simulink model "EvilSpagetty"  (R2020b)
settings: Solver=VariableStepAuto  StartTime=0.0  StopTime=3  RelTol=1e-3
(part 2 of 7)

== matlab function EvilSpagetty/Vt1 ==
  data: u1 input; y output; u2 input; u3 input; u4 input; u5 input; u6 input; u7 input; u8 input; u9 input; u10 input
function y = fcn(u1,u2,u3,u4,u5,u6,u7,u8,u9,u10)
theta1=u1;
theta2=u2;
theta3=u3;
theta4=u4;
theta5=u5;
d_theta1=u6;
d_theta2=u7;
d_theta3=u8;
d_theta4=u9;
d_theta5=u10;
Z=[(9004151162956663*d_theta2^2*cos(theta2 + theta3 + theta4 - theta5))/37778931862957161709568 - (6049849466133601*d_theta2^2*sin(theta2))/151115727451828646838272 + (3240011242931075*d_theta2^2*cos(theta2 + theta3 + theta4 - 2*theta5))/73786976294838206464 - (3240011242931075*d_theta2^2*cos(theta2 + theta3 + theta4 + 2*theta5))/73786976294838206464 + (9004151162956663*d_theta3^2*cos(theta2 + theta3 + theta4 - theta5))/37778931862957161709568 + (3240011242931075*d_theta3^2*cos(theta2 + theta3 + theta4 - 2*theta5))/73786976294838206464 - (3240011242931075*d_theta3^2*cos(theta2 + theta3 + theta4 + 2*theta5))/73786976294838206464 + (9004151162956663*d_theta4^2*cos(theta2 + theta3 + theta4 - theta5))/37778931862957161709568 + (3240011242931075*d_theta4^2*cos(theta2 + theta3 + theta4 - 2*theta5))/73786976294838206464 - (3240011242931075*d_theta4^2*cos(theta2 + theta3 + theta4 + 2*theta5))/73786976294838206464 - (9004151162956663*d_theta5^2*cos(theta2 + theta3 + theta4 - theta5))/37778931862957161709568 - (4653258611581729*d_theta2^2*sin(theta2 + theta3 + theta4 - theta5))/73786976294838206464 + (2282168433090971*d_theta2^2*sin(theta2 + theta3 + theta4 - 2*theta5))/37778931862957161709568 + (2282168433090971*d_theta2^2*sin(theta2 + theta3 + theta4 + 2*theta5))/37778931862957161709568 - (4653258611581729*d_theta3^2*sin(theta2 + theta3 + theta4 - theta5))/73786976294838206464 + (2282168433090971*d_theta3^2*sin(theta2 + theta3 + theta4 - 2*theta5))/37778931862957161709568 + (2282168433090971*d_theta3^2*sin(theta2 + theta3 + theta4 + 2*theta5))/37778931862957161709568 - (4653258611581729*d_theta4^2*sin(theta2 + theta3 + theta4 - theta5))/73786976294838206464 + (2282168433090971*d_theta4^2*sin(theta2 + theta3 + theta4 - 2*theta5))/37778931862957161709568 + (2282168433090971*d_theta4^2*sin(theta2 + theta3 + theta4 + 2*theta5))/37778931862957161709568 + (4653258611581729*d_theta5^2*sin(theta2 + theta3 + theta4 - theta5))/73786976294838206464 + (d_theta1*d_theta4)/2787593149816327892691964784081045188247552 + (5959870363491779*d_theta2^2*cos(theta2 - theta5))/4722366482869645213696 - (5959870363491779*d_theta5^2*cos(theta2 - theta5))/4722366482869645213696 - (8313573984755043*d_theta2^2*sin(theta2 - theta5))/18446744073709551616 + (8313573984755043*d_theta5^2*sin(theta2 - theta5))/18446744073709551616 - (2263187056021513*d_theta2^2*cos(theta2 + theta3 + theta4))/18446744073709551616 + (7988070105025833*d_theta2^2*cos(theta2 + theta3 + theta5))/9444732965739290427392 - (2263187056021513*d_theta3^2*cos(theta2 + theta3 + theta4))/18446744073709551616 + (7988070105025833*d_theta3^2*cos(theta2 + theta3 + theta5))/9444732965739290427392 - (2263187056021513*d_theta4^2*cos(theta2 + theta3 + theta4))/18446744073709551616 - (7988070105025833*d_theta5^2*cos(theta2 + theta3 + theta5))/9444732965739290427392 - (8356375065390427*d_theta2^2*sin(theta2 + theta3 + theta4))/9223372036854775808 + (5571380563941847*d_theta2^2*sin(theta2 + theta3 + theta5))/18446744073709551616 - (8356375065390427*d_theta3^2*sin(theta2 + theta3 + theta4))/9223372036854775808 + (5571380563941847*d_theta3^2*sin(theta2 + theta3 + theta5))/18446744073709551616 - (8356375065390427*d_theta4^2*sin(theta2 + theta3 + theta4))/9223372036854775808 - (5571380563941847*d_theta5^2*sin(theta2 + theta3 + theta5))/18446744073709551616 + (7988070105025833*d_theta2^2*cos(theta2 + theta3 - theta5))/9444732965739290427392 + (7988070105025833*d_theta3^2*cos(theta2 + theta3 - theta5))/9444732965739290427392 - (7988070105025833*d_theta5^2*cos(theta2 + theta3 - theta5))/9444732965739290427392 - (5571380563941847*d_theta2^2*sin(theta2 + theta3 - theta5))/18446744073709551616 - (5571380563941847*d_theta3^2*sin(theta2 + theta3 - theta5))/18446744073709551616 + (5571380563941847*d_theta5^2*sin(theta2 + theta3 - theta5))/18446744073709551616 + (9004151162956663*d_theta2^2*cos(theta2 + theta3 + theta4 + theta5))/37778931862957161709568 + (9004151162956663*d_theta3^2*cos(theta2 + theta3 + theta4 + theta5))/37778931862957161709568 + (9004151162956663*d_theta4^2*cos(theta2 + theta3 + theta4 + theta5))/37778931862957161709568 - (9004151162956663*d_theta5^2*cos(theta2 + theta3 + theta4 + theta5))/37778931862957161709568 + (4653258611581729*d_theta2^2*sin(theta2 + theta3 + theta4 + theta5))/73786976294838206464 + (4653258611581729*d_theta3^2*sin(theta2 + theta3 + theta4 + theta5))/73786976294838206464 + (4653258611581729*d_theta4^2*sin(theta2 + theta3 + theta4 + theta5))/73786976294838206464 - (4653258611581729*d_theta5^2*sin(theta2 + theta3 + theta4 + theta5))/73786976294838206464 - (8937783066759625*d_theta2^2*cos(theta2 + theta3))/4611686018427387904 - (8937783066759625*d_theta3^2*cos(theta2 + theta3))/4611686018427387904 + (5959870363491779*d_theta2^2*cos(theta2 + theta5))/4722366482869645213696 - (5959870363491779*d_theta5^2*cos(theta2 + theta5))/4722366482869645213696 - (581180430255771*d_theta2^2*sin(theta2 + theta3))/72057594037927936 - (581180430255771*d_theta3^2*sin(theta2 + theta3))/72057594037927936 + (8313573984755043*d_theta2^2*sin(theta2 + theta5))/18446744073709551616 - (8313573984755043*d_theta5^2*sin(theta2 + theta5))/18446744073709551616 - (5218682484910043*d_theta2^2*cos(theta2))/147573952589676412928 - (7028085605816175*d_theta1*d_theta3*cos(theta3))/590295810358705651712 - (d_theta1*d_theta2*cos(theta5))/5575186299632655785383929568162090376495104 - (d_theta1*d_theta3*cos(theta5))/5575186299632655785383929568162090376495104 - (d_theta1*d_theta4*cos(theta5))/5575186299632655785383929568162090376495104 + (12544169*d_theta1*d_theta2*cos(2*theta3 - 2*theta2 + theta5))/22300745198530623141535718272648361505980416 + (12544169*d_theta1*d_theta2*cos(2*theta2 - 2*theta3 + theta5))/22300745198530623141535718272648361505980416 - (1393797*d_theta1*d_theta2*cos(2*theta2 + 2*theta3 + theta5))/22300745198530623141535718272648361505980416 + (12544169*d_theta1*d_theta2*cos(2*theta4 - 2*theta2 + theta5))/22300745198530623141535718272648361505980416 + (12544169*d_theta1*d_theta2*cos(2*theta2 - 2*theta4 + theta5))/22300745198530623141535718272648361505980416 - (1393797*d_theta1*d_theta2*cos(2*theta2 + 2*theta4 + theta5))/22300745198530623141535718272648361505980416 + (12544169*d_theta1*d_theta3*cos(2*theta3 - 2*theta2 + theta5))/22300745198530623141535718272648361505980416 + (12544169*d_theta1*d_theta3*cos(2*theta2 - 2*theta3 + theta5))/22300745198530623141535718272648361505980416 - (1393797*d_theta1*d_theta3*cos(2*theta2 + 2*theta3 + theta5))/22300745198530623141535718272648361505980416 + (12544169*d_theta1*d_theta3*cos(2*theta4 - 2*theta3 + theta5))/22300745198530623141535718272648361505980416 + (12544169*d_theta1*d_theta3*cos(2*theta3 - 2*theta4 + theta5))/22300745198530623141535718272648361505980416 - (1393797*d_theta1*d_theta3*cos(2*theta3 + 2*theta4 + theta5))/22300745198530623141535718272648361505980416 + (12544169*d_theta1*d_theta4*cos(2*theta4 - 2*theta2 + theta5))/22300745198530623141535718272648361505980416 + (12544169*d_theta1*d_theta4*cos(2*theta2 - 2*theta4 + theta5))/22300745198530623141535718272648361505980416 - (1393797*d_theta1*d_theta4*cos(2*theta2 + 2*theta4 + theta5))/22300745198530623141535718272648361505980416 + (2787593*d_theta1*d_theta5*cos(2*theta2 + 2*theta3 + theta5))/11150372599265311570767859136324180752990208 + (12544169*d_theta1*d_theta4*cos(2*theta4 - 2*theta3 + theta5))/22300745198530623141535718272648361505980416 + (12544169*d_theta1*d_theta4*cos(2*theta3 - 2*theta4 + theta5))/22300745198530623141535718272648361505980416 - (1393797*d_theta1*d_theta4*cos(2*theta3 + 2*theta4 + theta5))/22300745198530623141535718272648361505980416 + (2787593*d_theta1*d_theta5*cos(2*theta2 + 2*theta4 + theta5))/11150372599265311570767859136324180752990208 + (2787593*d_theta1*d_theta5*cos(2*theta3 + 2*theta4 + theta5))/11150372599265311570767859136324180752990208 - (d_theta1*d_theta2*sin(theta4))/696898287454081973172991196020261297061888 - (3257081095467945*d_theta1*d_theta3*sin(theta3))/288230376151711744 - (d_theta1*d_theta3*sin(theta4))/696898287454081973172991196020261297061888 - (7220698343344529*d_theta1*d_theta4*sin(theta4))/2305843009213693952 + (d_theta1*d_theta2*sin(2*theta2 + theta3 - theta4))/1393796574908163946345982392040522594123776 + (d_theta1*d_theta2*sin(2*theta2 - theta3 + theta4))/1393796574908163946345982392040522594123776 - (7220698343344529*d_theta1*d_theta2*sin(2*theta2 + 2*theta3 + theta4))/1152921504606846976 + (7136239*d_theta1*d_theta2*sin(2*theta2 + theta4 - theta5))/5708990770823839524233143877797980545530986496 + (21408715*d_theta1*d_theta2*sin(2*theta2 - theta4 + theta5))/5708990770823839524233143877797980545530986496 - (7220698343344529*d_theta1*d_theta3*sin(2*theta2 + 2*theta3 + theta4))/1152921504606846976 - (7220698343344529*d_theta1*d_theta4*sin(2*theta2 + 2*theta3 + theta4))/2305843009213693952 + (7136239*d_theta1*d_theta3*sin(2*theta3 + theta4 - theta5))/5708990770823839524233143877797980545530986496 + (21408715*d_theta1*d_theta3*sin(2*theta3 - theta4 + theta5))/5708990770823839524233143877797980545530986496 - (3568119*d_theta1*d_theta4*sin(2*theta2 + theta4 - theta5))/2854495385411919762116571938898990272765493248 - (3568119*d_theta1*d_theta4*sin(2*theta3 + theta4 - theta5))/2854495385411919762116571938898990272765493248 + (3568119*d_theta1*d_theta5*sin(2*theta2 + theta4 - theta5))/2854495385411919762116571938898990272765493248 + (3568119*d_theta1*d_theta5*sin(2*theta3 + theta4 - theta5))/2854495385411919762116571938898990272765493248 + (8313573984755043*d_theta1*d_theta2*cos(2*theta2 + theta3 + theta4 + theta5))/9223372036854775808 + (8313573984755043*d_theta1*d_theta3*cos(2*theta2 + theta3 + theta4 + theta5))/18446744073709551616 + (9004151162956663*d_theta2*d_theta3*cos(theta2 + theta3 + theta4 - theta5))/18889465931478580854784 + (8313573984755043*d_theta1*d_theta4*cos(2*theta2 + theta3 + theta4 + theta5))/18446744073709551616 + (3240011242931075*d_theta2*d_theta3*cos(theta2 + theta3 + theta4 - 2*theta5))/36893488147419103232 - (3240011242931075*d_theta2*d_theta3*cos(theta2 + theta3 + theta4 + 2*theta5))/36893488147419103232 + (9004151162956663*d_theta2*d_theta4*cos(theta2 + theta3 + theta4 - theta5))/18889465931478580854784 + (8313573984755043*d_theta1*d_theta5*cos(2*theta2 + theta3 + theta4 + theta5))/18446744073709551616 + (3240011242931075*d_theta2*d_theta4*cos(theta2 + theta3 + theta4 - 2*theta5))/36893488147419103232 - (3240011242931075*d_theta2*d_theta4*cos(theta2 + theta3 + theta4 + 2*theta5))/36893488147419103232 + (9004151162956663*d_theta3*d_theta4*cos(theta2 + theta3 + theta4 - theta5))/18889465931478580854784 - (3240011242931075*d_theta2*d_theta5*cos(theta2 + theta3 + theta4 - 2*theta5))/36893488147419103232 - (3240011242931075*d_theta2*d_theta5*cos(theta2 + theta3 + theta4 + 2*theta5))/36893488147419103232 + (3240011242931075*d_theta3*d_theta4*cos(theta2 + theta3 + theta4 - 2*theta5))/36893488147419103232 - (3240011242931075*d_theta3*d_theta4*cos(theta2 + theta3 + theta4 + 2*theta5))/36893488147419103232 - (3240011242931075*d_theta3*d_theta5*cos(theta2 + theta3 + theta4 - 2*theta5))/36893488147419103232 - (3240011242931075*d_theta3*d_theta5*cos(theta2 + theta3 + theta4 + 2*theta5))/36893488147419103232 - (3240011242931075*d_theta4*d_theta5*cos(theta2 + theta3 + theta4 - 2*theta5))/36893488147419103232 - (3240011242931075*d_theta4*d_theta5*cos(theta2 + theta3 + theta4 + 2*theta5))/36893488147419103232 - (5959870363491779*d_theta1*d_theta2*sin(2*theta2 + theta3 + theta4 + theta5))/2361183241434822606848 - (5959870363491779*d_theta1*d_theta3*sin(2*theta2 + theta3 + theta4 + theta5))/4722366482869645213696 - (4653258611581729*d_theta2*d_theta3*sin(theta2 + theta3 + theta4 - theta5))/36893488147419103232 - (5959870363491779*d_theta1*d_theta4*sin(2*theta2 + theta3 + theta4 + theta5))/4722366482869645213696 + (2282168433090971*d_theta2*d_theta3*sin(theta2 + theta3 + theta4 - 2*theta5))/18889465931478580854784 + (2282168433090971*d_theta2*d_theta3*sin(theta2 + theta3 + theta4 + 2*theta5))/18889465931478580854784 - (4653258611581729*d_theta2*d_theta4*sin(theta2 + theta3 + theta4 - theta5))/36893488147419103232 - (5959870363491779*d_theta1*d_theta5*sin(2*theta2 + theta3 + theta4 + theta5))/4722366482869645213696 + (2282168433090971*d_theta2*d_theta4*sin(theta2 + theta3 + theta4 - 2*theta5))/18889465931478580854784 + (2282168433090971*d_theta2*d_theta4*sin(theta2 + theta3 + theta4 + 2*theta5))/18889465931478580854784 - (4653258611581729*d_theta3*d_theta4*sin(theta2 + theta3 + theta4 - theta5))/36893488147419103232 - (2282168433090971*d_theta2*d_theta5*sin(theta2 + theta3 + theta4 - 2*theta5))/18889465931478580854784 + (2282168433090971*d_theta2*d_theta5*sin(theta2 + theta3 + theta4 + 2*theta5))/18889465931478580854784 + (2282168433090971*d_theta3*d_theta4*sin(theta2 + theta3 + theta4 - 2*theta5))/18889465931478580854784 + (2282168433090971*d_theta3*d_theta4*sin(theta2 + theta3 + theta4 + 2*theta5))/18889465931478580854784 - (2282168433090971*d_theta3*d_theta5*sin(theta2 + theta3 + theta4 - 2*theta5))/18889465931478580854784 + (2282168433090971*d_theta3*d_theta5*sin(theta2 + theta3 + theta4 + 2*theta5))/18889465931478580854784 - (2282168433090971*d_theta4*d_theta5*sin(theta2 + theta3 + theta4 - 2*theta5))/18889465931478580854784 + (2282168433090971*d_theta4*d_theta5*sin(theta2 + theta3 + theta4 + 2*theta5))/18889465931478580854784 - (7028085605816175*d_theta1*d_theta2*cos(2*theta2 + theta3))/295147905179352825856 - (7028085605816175*d_theta1*d_theta3*cos(2*theta2 + theta3))/590295810358705651712 + (2787593*d_theta1*d_theta2*cos(2*theta2 + theta5))/5575186299632655785383929568162090376495104 + (2787593*d_theta1*d_theta3*cos(2*theta3 + theta5))/5575186299632655785383929568162090376495104 + (5571380563941847*d_theta1*d_theta4*cos(theta4 - theta5))/18446744073709551616 + (2787593*d_theta1*d_theta5*cos(2*theta2 + theta5))/11150372599265311570767859136324180752990208 + (2787593*d_theta1*d_theta4*cos(2*theta4 + theta5))/5575186299632655785383929568162090376495104 - (5571380563941847*d_theta1*d_theta5*cos(theta4 - theta5))/18446744073709551616 + (2787593*d_theta1*d_theta5*cos(2*theta3 + theta5))/11150372599265311570767859136324180752990208 + (2787593*d_theta1*d_theta5*cos(2*theta4 + theta5))/11150372599265311570767859136324180752990208 + (d_theta1*d_theta2*cos(2*theta2 - 2*theta3 + 2*theta4 - theta5))/89202980794122492566142873090593446023921664 + (d_theta1*d_theta2*cos(2*theta2 + 2*theta3 - 2*theta4 - theta5))/89202980794122492566142873090593446023921664 + (4653258611581729*d_theta1*d_theta2*cos(2*theta2 + 2*theta3 + 2*theta4 - theta5))/36893488147419103232 - (2282168433090971*d_theta1*d_theta2*cos(2*theta2 + 2*theta3 + 2*theta4 - 2*theta5))/37778931862957161709568 + (2282168433090971*d_theta1*d_theta2*cos(2*theta2 + 2*theta3 + 2*theta4 + 2*theta5))/37778931862957161709568 + (22300745*d_theta1*d_theta3*cos(2*theta2 - 2*theta3 + 2*theta4 - theta5))/44601490397061246283071436545296723011960832 + (d_theta1*d_theta3*cos(2*theta2 + 2*theta3 - 2*theta4 - theta5))/89202980794122492566142873090593446023921664 + (4653258611581729*d_theta1*d_theta3*cos(2*theta2 + 2*theta3 + 2*theta4 - theta5))/36893488147419103232 - (2282168433090971*d_theta1*d_theta3*cos(2*theta2 + 2*theta3 + 2*theta4 - 2*theta5))/37778931862957161709568 + (2282168433090971*d_theta1*d_theta3*cos(2*theta2 + 2*theta3 + 2*theta4 + 2*theta5))/37778931862957161709568 + (d_theta1*d_theta4*cos(2*theta2 - 2*theta3 + 2*theta4 - theta5))/89202980794122492566142873090593446023921664 + (22300745*d_theta1*d_theta4*cos(2*theta2 + 2*theta3 - 2*theta4 - theta5))/44601490397061246283071436545296723011960832 + (4653258611581729*d_theta1*d_theta4*cos(2*theta2 + 2*theta3 + 2*theta4 - theta5))/36893488147419103232 - (2282168433090971*d_theta1*d_theta4*cos(2*theta2 + 2*theta3 + 2*theta4 - 2*theta5))/37778931862957161709568 + (2282168433090971*d_theta1*d_theta4*cos(2*theta2 + 2*theta3 + 2*theta4 + 2*theta5))/37778931862957161709568 - (4653258611581729*d_theta1*d_theta5*cos(2*theta2 + 2*theta3 + 2*theta4 - theta5))/73786976294838206464 + (2282168433090971*d_theta1*d_theta5*cos(2*theta2 + 2*theta3 + 2*theta4 - 2*theta5))/37778931862957161709568 + (2282168433090971*d_theta1*d_theta5*cos(2*theta2 + 2*theta3 + 2*theta4 + 2*theta5))/37778931862957161709568 - (3257081095467945*d_theta1*d_theta2*sin(2*theta2 + theta3))/144115188075855872 + (6968983*d_theta1*d_theta2*sin(2*theta2 + theta4))/1393796574908163946345982392040522594123776 - (3257081095467945*d_theta1*d_theta3*sin(2*theta2 + theta3))/288230376151711744 - (2854495*d_theta1*d_theta2*sin(2*theta2 + theta5))/5708990770823839524233143877797980545530986496 + (6968983*d_theta1*d_theta3*sin(2*theta3 + theta4))/1393796574908163946345982392040522594123776 + (6968983*d_theta1*d_theta4*sin(2*theta2 + theta4))/1393796574908163946345982392040522594123776 - (2854495*d_theta1*d_theta3*sin(2*theta3 + theta5))/5708990770823839524233143877797980545530986496 + (6968983*d_theta1*d_theta4*sin(2*theta3 + theta4))/1393796574908163946345982392040522594123776 + (7988070105025833*d_theta1*d_theta4*sin(theta4 - theta5))/9444732965739290427392 - (2854495*d_theta1*d_theta5*sin(2*theta2 + theta5))/11417981541647679048466287755595961091061972992 - (2854495*d_theta1*d_theta4*sin(2*theta4 + theta5))/5708990770823839524233143877797980545530986496 - (7988070105025833*d_theta1*d_theta5*sin(theta4 - theta5))/9444732965739290427392 - (2854495*d_theta1*d_theta5*sin(2*theta3 + theta5))/11417981541647679048466287755595961091061972992 - (2854495*d_theta1*d_theta5*sin(2*theta4 + theta5))/11417981541647679048466287755595961091061972992 - (2263187056021513*d_theta2*d_theta3*cos(theta2 + theta3 + theta4))/9223372036854775808 + (7988070105025833*d_theta2*d_theta3*cos(theta2 + theta3 + theta5))/4722366482869645213696 - (2263187056021513*d_theta2*d_theta4*cos(theta2 + theta3 + theta4))/9223372036854775808 + (8313573984755043*d_theta1*d_theta3*cos(theta3 + theta4 + theta5))/18446744073709551616 + (1951319518623669*d_theta2*d_theta5*cos(theta2 + theta3 + theta4))/9223372036854775808 - (2263187056021513*d_theta3*d_theta4*cos(theta2 + theta3 + theta4))/9223372036854775808 + (8313573984755043*d_theta1*d_theta4*cos(theta3 + theta4 + theta5))/18446744073709551616 + (1951319518623669*d_theta3*d_theta5*cos(theta2 + theta3 + theta4))/9223372036854775808 + (8313573984755043*d_theta1*d_theta5*cos(theta3 + theta4 + theta5))/18446744073709551616 + (1951319518623669*d_theta4*d_theta5*cos(theta2 + theta3 + theta4))/9223372036854775808 - (d_theta1*d_theta2*sin(2*theta2 + 2*theta3 - theta4 - theta5))/5708990770823839524233143877797980545530986496 + (9004151162956663*d_theta1*d_theta2*sin(2*theta2 + 2*theta3 + 2*theta4 - theta5))/18889465931478580854784 - (d_theta1*d_theta3*sin(2*theta2 + 2*theta3 - theta4 - theta5))/5708990770823839524233143877797980545530986496 - (4460149*d_theta1*d_theta2*sin(2*theta3 - 2*theta2 + 2*theta4 + 2*theta5))/89202980794122492566142873090593446023921664 + (4460149*d_theta1*d_theta2*sin(2*theta2 - 2*theta3 - 2*theta4 + 2*theta5))/89202980794122492566142873090593446023921664 + (3240011242931075*d_theta1*d_theta2*sin(2*theta2 + 2*theta3 + 2*theta4 - 2*theta5))/73786976294838206464 + (3240011242931075*d_theta1*d_theta2*sin(2*theta2 + 2*theta3 + 2*theta4 + 2*theta5))/73786976294838206464 + (9004151162956663*d_theta1*d_theta3*sin(2*theta2 + 2*theta3 + 2*theta4 - theta5))/18889465931478580854784 - (4460149*d_theta1*d_theta3*sin(2*theta2 - 2*theta3 + 2*theta4 - 2*theta5))/89202980794122492566142873090593446023921664 - (4460149*d_theta1*d_theta3*sin(2*theta2 - 2*theta3 + 2*theta4 + 2*theta5))/89202980794122492566142873090593446023921664 + (3240011242931075*d_theta1*d_theta3*sin(2*theta2 + 2*theta3 + 2*theta4 - 2*theta5))/73786976294838206464 + (3240011242931075*d_theta1*d_theta3*sin(2*theta2 + 2*theta3 + 2*theta4 + 2*theta5))/73786976294838206464 + (9004151162956663*d_theta1*d_theta4*sin(2*theta2 + 2*theta3 + 2*theta4 - theta5))/18889465931478580854784 - (4460149*d_theta1*d_theta4*sin(2*theta2 + 2*theta3 - 2*theta4 - 2*theta5))/89202980794122492566142873090593446023921664 - (4460149*d_theta1*d_theta4*sin(2*theta2 + 2*theta3 - 2*theta4 + 2*theta5))/89202980794122492566142873090593446023921664 + (3240011242931075*d_theta1*d_theta4*sin(2*theta2 + 2*theta3 + 2*theta4 - 2*theta5))/73786976294838206464 + (3240011242931075*d_theta1*d_theta4*sin(2*theta2 + 2*theta3 + 2*theta4 + 2*theta5))/73786976294838206464 - (9004151162956663*d_theta1*d_theta5*sin(2*theta2 + 2*theta3 + 2*theta4 - theta5))/37778931862957161709568 - (3240011242931075*d_theta1*d_theta5*sin(2*theta2 + 2*theta3 + 2*theta4 - 2*theta5))/73786976294838206464 + (3240011242931075*d_theta1*d_theta5*sin(2*theta2 + 2*theta3 + 2*theta4 + 2*theta5))/73786976294838206464 - (8356375065390427*d_theta2*d_theta3*sin(theta2 + theta3 + theta4))/4611686018427387904 + (5571380563941847*d_theta2*d_theta3*sin(theta2 + theta3 + theta5))/9223372036854775808 - (8356375065390427*d_theta2*d_theta4*sin(theta2 + theta3 + theta4))/4611686018427387904 - (5959870363491779*d_theta1*d_theta3*sin(theta3 + theta4 + theta5))/4722366482869645213696 - (8356375065390427*d_theta3*d_theta4*sin(theta2 + theta3 + theta4))/4611686018427387904 - (5959870363491779*d_theta1*d_theta4*sin(theta3 + theta4 + theta5))/4722366482869645213696 - (5959870363491779*d_theta1*d_theta5*sin(theta3 + theta4 + theta5))/4722366482869645213696 + (3825825015716409*d_theta1*d_theta2*cos(2*theta2))/73786976294838206464 + (d_theta1*d_theta5*cos(2*theta2))/5708990770823839524233143877797980545530986496 + (d_theta1*d_theta5*cos(2*theta3))/5708990770823839524233143877797980545530986496 + (d_theta1*d_theta5*cos(2*theta4))/5708990770823839524233143877797980545530986496 + (2282168433090971*d_theta1*d_theta5*cos(2*theta5))/18889465931478580854784 - (2695991646372651*d_theta1*d_theta2*cos(2*theta2 + 2*theta3 + 2*theta4))/4611686018427387904 - (1393797*d_theta1*d_theta2*cos(2*theta2 + 2*theta3 - theta5))/22300745198530623141535718272648361505980416 + (5708989*d_theta1*d_theta2*cos(2*theta2 + 2*theta3 - 2*theta5))/91343852333181432387730302044767688728495783936 - (5708989*d_theta1*d_theta2*cos(2*theta2 + 2*theta3 + 2*theta5))/91343852333181432387730302044767688728495783936 - (1393797*d_theta1*d_theta2*cos(2*theta2 + 2*theta4 - theta5))/22300745198530623141535718272648361505980416 - (2695991646372651*d_theta1*d_theta3*cos(2*theta2 + 2*theta3 + 2*theta4))/4611686018427387904 - (1393797*d_theta1*d_theta3*cos(2*theta2 + 2*theta3 - theta5))/22300745198530623141535718272648361505980416 + (5708989*d_theta1*d_theta2*cos(2*theta2 + 2*theta4 - 2*theta5))/91343852333181432387730302044767688728495783936 - (5708989*d_theta1*d_theta2*cos(2*theta2 + 2*theta4 + 2*theta5))/91343852333181432387730302044767688728495783936 + (5708989*d_theta1*d_theta3*cos(2*theta2 + 2*theta3 - 2*theta5))/91343852333181432387730302044767688728495783936 - (5708989*d_theta1*d_theta3*cos(2*theta2 + 2*theta3 + 2*theta5))/91343852333181432387730302044767688728495783936 - (2695991646372651*d_theta1*d_theta4*cos(2*theta2 + 2*theta3 + 2*theta4))/4611686018427387904 - (1393797*d_theta1*d_theta3*cos(2*theta3 + 2*theta4 - theta5))/22300745198530623141535718272648361505980416 - (1393797*d_theta1*d_theta4*cos(2*theta2 + 2*theta4 - theta5))/22300745198530623141535718272648361505980416 - (d_theta1*d_theta5*cos(2*theta3 - 2*theta2 + 2*theta4))/45671926166590716193865151022383844364247891968 - (d_theta1*d_theta5*cos(2*theta2 - 2*theta3 + 2*theta4))/45671926166590716193865151022383844364247891968 - (d_theta1*d_theta5*cos(2*theta2 + 2*theta3 - 2*theta4))/45671926166590716193865151022383844364247891968 - (d_theta1*d_theta5*cos(2*theta2 + 2*theta3 + 2*theta4))/45671926166590716193865151022383844364247891968 - (2787593*d_theta1*d_theta5*cos(2*theta2 + 2*theta3 - theta5))/11150372599265311570767859136324180752990208 + (5708989*d_theta1*d_theta3*cos(2*theta3 + 2*theta4 - 2*theta5))/91343852333181432387730302044767688728495783936 - (5708989*d_theta1*d_theta3*cos(2*theta3 + 2*theta4 + 2*theta5))/91343852333181432387730302044767688728495783936 + (5708989*d_theta1*d_theta4*cos(2*theta2 + 2*theta4 - 2*theta5))/91343852333181432387730302044767688728495783936 - (5708989*d_theta1*d_theta4*cos(2*theta2 + 2*theta4 + 2*theta5))/91343852333181432387730302044767688728495783936 - (1393797*d_theta1*d_theta4*cos(2*theta3 + 2*theta4 - theta5))/22300745198530623141535718272648361505980416 + (d_theta1*d_theta5*cos(2*theta3 - 2*theta2 + 2*theta5))/91343852333181432387730302044767688728495783936 + (d_theta1*d_theta5*cos(2*theta2 - 2*theta3 + 2*theta5))/91343852333181432387730302044767688728495783936 - (2854495*d_theta1*d_theta5*cos(2*theta2 + 2*theta3 - 2*theta5))/45671926166590716193865151022383844364247891968 - (2854495*d_theta1*d_theta5*cos(2*theta2 + 2*theta3 + 2*theta5))/45671926166590716193865151022383844364247891968 - (2787593*d_theta1*d_theta5*cos(2*theta2 + 2*theta4 - theta5))/11150372599265311570767859136324180752990208 + (5708989*d_theta1*d_theta4*cos(2*theta3 + 2*theta4 - 2*theta5))/91343852333181432387730302044767688728495783936 - (5708989*d_theta1*d_theta4*cos(2*theta3 + 2*theta4 + 2*theta5))/91343852333181432387730302044767688728495783936 + (d_theta1*d_theta5*cos(2*theta4 - 2*theta2 + 2*theta5))/91343852333181432387730302044767688728495783936 + (d_theta1*d_theta5*cos(2*theta2 - 2*theta4 + 2*theta5))/91343852333181432387730302044767688728495783936 - (2854495*d_theta1*d_theta5*cos(2*theta2 + 2*theta4 - 2*theta5))/45671926166590716193865151022383844364247891968 - (2854495*d_theta1*d_theta5*cos(2*theta2 + 2*theta4 + 2*theta5))/45671926166590716193865151022383844364247891968 - (2787593*d_theta1*d_theta5*cos(2*theta3 + 2*theta4 - theta5))/11150372599265311570767859136324180752990208 + (d_theta1*d_theta5*cos(2*theta4 - 2*theta3 + 2*theta5))/91343852333181432387730302044767688728495783936 + (d_theta1*d_theta5*cos(2*theta3 - 2*theta4 + 2*theta5))/91343852333181432387730302044767688728495783936 - (2854495*d_theta1*d_theta5*cos(2*theta3 + 2*theta4 - 2*theta5))/45671926166590716193865151022383844364247891968 - (2854495*d_theta1*d_theta5*cos(2*theta3 + 2*theta4 + 2*theta5))/45671926166590716193865151022383844364247891968 - (4725330594848641*d_theta1*d_theta2*sin(2*theta2))/144115188075855872 - (d_theta1*d_theta2*sin(2*theta3))/44601490397061246283071436545296723011960832 - (d_theta1*d_theta3*sin(2*theta2))/44601490397061246283071436545296723011960832 - (d_theta1*d_theta2*sin(2*theta4))/44601490397061246283071436545296723011960832 + (61327049*d_theta1*d_theta3*sin(2*theta3))/44601490397061246283071436545296723011960832 - (d_theta1*d_theta4*sin(2*theta2))/44601490397061246283071436545296723011960832 - (d_theta1*d_theta3*sin(2*theta4))/44601490397061246283071436545296723011960832 - (d_theta1*d_theta4*sin(2*theta3))/44601490397061246283071436545296723011960832 + (61327057*d_theta1*d_theta4*sin(2*theta4))/44601490397061246283071436545296723011960832 + (3240011242931075*d_theta1*d_theta5*sin(2*theta5))/36893488147419103232 - (11150373*d_theta1*d_theta2*sin(2*theta3 - 2*theta2 + 2*theta4))/11150372599265311570767859136324180752990208 - (d_theta1*d_theta2*sin(2*theta2 - 2*theta3 + 2*theta4))/22300745198530623141535718272648361505980416 - (d_theta1*d_theta2*sin(2*theta2 + 2*theta3 - 2*theta4))/22300745198530623141535718272648361505980416 - (1160499590055099*d_theta1*d_theta2*sin(2*theta2 + 2*theta3 + 2*theta4))/2305843009213693952 - (2787593*d_theta1*d_theta2*sin(2*theta3 - 2*theta2 + 2*theta5))/89202980794122492566142873090593446023921664 + (5575185*d_theta1*d_theta2*sin(2*theta2 - 2*theta3 + 2*theta5))/178405961588244985132285746181186892047843328 + (8362779*d_theta1*d_theta2*sin(2*theta2 + 2*theta3 - 2*theta5))/89202980794122492566142873090593446023921664 + (8362779*d_theta1*d_theta2*sin(2*theta2 + 2*theta3 + 2*theta5))/89202980794122492566142873090593446023921664 - (d_theta1*d_theta3*sin(2*theta3 - 2*theta2 + 2*theta4))/22300745198530623141535718272648361505980416 - (11150373*d_theta1*d_theta3*sin(2*theta2 - 2*theta3 + 2*theta4))/11150372599265311570767859136324180752990208 - (d_theta1*d_theta3*sin(2*theta2 + 2*theta3 - 2*theta4))/22300745198530623141535718272648361505980416 - (1160499590055099*d_theta1*d_theta3*sin(2*theta2 + 2*theta3 + 2*theta4))/2305843009213693952 - (2787593*d_theta1*d_theta2*sin(2*theta4 - 2*theta2 + 2*theta5))/89202980794122492566142873090593446023921664 + (5575185*d_theta1*d_theta2*sin(2*theta2 - 2*theta4 + 2*theta5))/178405961588244985132285746181186892047843328 + (8362779*d_theta1*d_theta2*sin(2*theta2 + 2*theta4 - 2*theta5))/89202980794122492566142873090593446023921664 + (8362779*d_theta1*d_theta2*sin(2*theta2 + 2*theta4 + 2*theta5))/89202980794122492566142873090593446023921664 + (5575185*d_theta1*d_theta3*sin(2*theta3 - 2*theta2 + 2*theta5))/178405961588244985132285746181186892047843328 - (2787593*d_theta1*d_theta3*sin(2*theta2 - 2*theta3 + 2*theta5))/89202980794122492566142873090593446023921664 + (8362779*d_theta1*d_theta3*sin(2*theta2 + 2*theta3 - 2*theta5))/89202980794122492566142873090593446023921664 + (8362779*d_theta1*d_theta3*sin(2*theta2 + 2*theta3 + 2*theta5))/89202980794122492566142873090593446023921664 - (d_theta1*d_theta4*sin(2*theta3 - 2*theta2 + 2*theta4))/22300745198530623141535718272648361505980416 - (d_theta1*d_theta4*sin(2*theta2 - 2*theta3 + 2*theta4))/22300745198530623141535718272648361505980416 - (11150373*d_theta1*d_theta4*sin(2*theta2 + 2*theta3 - 2*theta4))/11150372599265311570767859136324180752990208 - (1160499590055099*d_theta1*d_theta4*sin(2*theta2 + 2*theta3 + 2*theta4))/2305843009213693952 - (2787593*d_theta1*d_theta3*sin(2*theta4 - 2*theta3 + 2*theta5))/89202980794122492566142873090593446023921664 + (5575185*d_theta1*d_theta3*sin(2*theta3 - 2*theta4 + 2*theta5))/178405961588244985132285746181186892047843328 + (8362779*d_theta1*d_theta3*sin(2*theta3 + 2*theta4 - 2*theta5))/89202980794122492566142873090593446023921664 + (8362779*d_theta1*d_theta3*sin(2*theta3 + 2*theta4 + 2*theta5))/89202980794122492566142873090593446023921664 + (5575185*d_theta1*d_theta4*sin(2*theta4 - 2*theta2 + 2*theta5))/178405961588244985132285746181186892047843328 - (2787593*d_theta1*d_theta4*sin(2*theta2 - 2*theta4 + 2*theta5))/89202980794122492566142873090593446023921664 + (8362779*d_theta1*d_theta4*sin(2*theta2 + 2*theta4 - 2*theta5))/89202980794122492566142873090593446023921664 + (8362779*d_theta1*d_theta4*sin(2*theta2 + 2*theta4 + 2*theta5))/89202980794122492566142873090593446023921664 - (2787593*d_theta1*d_theta5*sin(2*theta2 + 2*theta3 - 2*theta5))/22300745198530623141535718272648361505980416 + (2787593*d_theta1*d_theta5*sin(2*theta2 + 2*theta3 + 2*theta5))/22300745198530623141535718272648361505980416 + (5575185*d_theta1*d_theta4*sin(2*theta4 - 2*theta3 + 2*theta5))/178405961588244985132285746181186892047843328 - (2787593*d_theta1*d_theta4*sin(2*theta3 - 2*theta4 + 2*theta5))/89202980794122492566142873090593446023921664 + (8362779*d_theta1*d_theta4*sin(2*theta3 + 2*theta4 - 2*theta5))/89202980794122492566142873090593446023921664 + (8362779*d_theta1*d_theta4*sin(2*theta3 + 2*theta4 + 2*theta5))/89202980794122492566142873090593446023921664 - (2787593*d_theta1*d_theta5*sin(2*theta2 + 2*theta4 - 2*theta5))/22300745198530623141535718272648361505980416 + (2787593*d_theta1*d_theta5*sin(2*theta2 + 2*theta4 + 2*theta5))/22300745198530623141535718272648361505980416 - (2787593*d_theta1*d_theta5*sin(2*theta3 + 2*theta4 - 2*theta5))/22300745198530623141535718272648361505980416 + (2787593*d_theta1*d_theta5*sin(2*theta3 + 2*theta4 + 2*theta5))/22300745198530623141535718272648361505980416 + (8313573984755043*d_theta1*d_theta2*cos(2*theta2 + theta3 + theta4 - theta5))/9223372036854775808 + (5571380563941847*d_theta1*d_theta2*cos(2*theta2 + 2*theta3 + theta4 + theta5))/9223372036854775808 + (8313573984755043*d_theta1*d_theta3*cos(2*theta2 + theta3 + theta4 - theta5))/18446744073709551616 + (5571380563941847*d_theta1*d_theta3*cos(2*theta2 + 2*theta3 + theta4 + theta5))/9223372036854775808 + (8313573984755043*d_theta1*d_theta4*cos(2*theta2 + theta3 + theta4 - theta5))/18446744073709551616 + (5571380563941847*d_theta1*d_theta4*cos(2*theta2 + 2*theta3 + theta4 + theta5))/18446744073709551616 - (8313573984755043*d_theta1*d_theta5*cos(2*theta2 + theta3 + theta4 - theta5))/18446744073709551616 + (5571380563941847*d_theta1*d_theta5*cos(2*theta2 + 2*theta3 + theta4 + theta5))/18446744073709551616 + (5959870363491779*d_theta1*d_theta2*sin(2*theta2 + theta3 + theta4 - theta5))/2361183241434822606848 - (d_theta1*d_theta2*sin(2*theta2 - 2*theta3 + theta4 + theta5))/5708990770823839524233143877797980545530986496 - (7988070105025833*d_theta1*d_theta2*sin(2*theta2 + 2*theta3 + theta4 + theta5))/4722366482869645213696 + (5959870363491779*d_theta1*d_theta3*sin(2*theta2 + theta3 + theta4 - theta5))/4722366482869645213696 - (7988070105025833*d_theta1*d_theta3*sin(2*theta2 + 2*theta3 + theta4 + theta5))/4722366482869645213696 + (5959870363491779*d_theta1*d_theta4*sin(2*theta2 + theta3 + theta4 - theta5))/4722366482869645213696 - (7988070105025833*d_theta1*d_theta4*sin(2*theta2 + 2*theta3 + theta4 + theta5))/9444732965739290427392 - (5959870363491779*d_theta1*d_theta5*sin(2*theta2 + theta3 + theta4 - theta5))/4722366482869645213696 - (7988070105025833*d_theta1*d_theta5*sin(2*theta2 + 2*theta3 + theta4 + theta5))/9444732965739290427392 - (1007824040173657*d_theta1*d_theta2*cos(2*theta2 + 2*theta3))/144115188075855872 + (2787593*d_theta1*d_theta2*cos(2*theta2 - theta5))/5575186299632655785383929568162090376495104 - (1007824040173657*d_theta1*d_theta3*cos(2*theta2 + 2*theta3))/144115188075855872 + (d_theta1*d_theta2*cos(2*theta3 - 2*theta5))/45671926166590716193865151022383844364247891968 + (d_theta1*d_theta2*cos(2*theta3 + 2*theta5))/45671926166590716193865151022383844364247891968 + (d_theta1*d_theta3*cos(2*theta2 - 2*theta5))/45671926166590716193865151022383844364247891968 + (d_theta1*d_theta3*cos(2*theta2 + 2*theta5))/45671926166590716193865151022383844364247891968 + (2787593*d_theta1*d_theta3*cos(2*theta3 - theta5))/5575186299632655785383929568162090376495104 + (d_theta1*d_theta2*cos(2*theta4 - 2*theta5))/45671926166590716193865151022383844364247891968 + (d_theta1*d_theta2*cos(2*theta4 + 2*theta5))/45671926166590716193865151022383844364247891968 + (d_theta1*d_theta4*cos(2*theta2 - 2*theta5))/45671926166590716193865151022383844364247891968 + (d_theta1*d_theta4*cos(2*theta2 + 2*theta5))/45671926166590716193865151022383844364247891968 - (2787593*d_theta1*d_theta5*cos(2*theta2 - theta5))/11150372599265311570767859136324180752990208 + (d_theta1*d_theta3*cos(2*theta4 - 2*theta5))/45671926166590716193865151022383844364247891968 + (d_theta1*d_theta3*cos(2*theta4 + 2*theta5))/45671926166590716193865151022383844364247891968 + (d_theta1*d_theta4*cos(2*theta3 - 2*theta5))/45671926166590716193865151022383844364247891968 + (d_theta1*d_theta4*cos(2*theta3 + 2*theta5))/45671926166590716193865151022383844364247891968 + (2787593*d_theta1*d_theta4*cos(2*theta4 - theta5))/5575186299632655785383929568162090376495104 - (8563485*d_theta1*d_theta5*cos(2*theta2 - 2*theta5))/45671926166590716193865151022383844364247891968 - (8563485*d_theta1*d_theta5*cos(2*theta2 + 2*theta5))/45671926166590716193865151022383844364247891968 - (2787593*d_theta1*d_theta5*cos(2*theta3 - theta5))/11150372599265311570767859136324180752990208 - (8563485*d_theta1*d_theta5*cos(2*theta3 - 2*theta5))/45671926166590716193865151022383844364247891968 - (8563485*d_theta1*d_theta5*cos(2*theta3 + 2*theta5))/45671926166590716193865151022383844364247891968 - (2787593*d_theta1*d_theta5*cos(2*theta4 - theta5))/11150372599265311570767859136324180752990208 - (8563485*d_theta1*d_theta5*cos(2*theta4 - 2*theta5))/45671926166590716193865151022383844364247891968 - (8563485*d_theta1*d_theta5*cos(2*theta4 + 2*theta5))/45671926166590716193865151022383844364247891968 + (8356542075167085*d_theta1*d_theta2*sin(2*theta2 + 2*theta3))/1152921504606846976 - (871123*d_theta1*d_theta2*sin(2*theta2 - theta4))/174224571863520493293247799005065324265472 + (61327057*d_theta1*d_theta2*sin(2*theta2 - 2*theta4))/89202980794122492566142873090593446023921664 + (36238715*d_theta1*d_theta2*sin(2*theta2 + 2*theta4))/44601490397061246283071436545296723011960832 + (2854495*d_theta1*d_theta2*sin(2*theta2 - theta5))/5708990770823839524233143877797980545530986496 + (8356542075167085*d_theta1*d_theta3*sin(2*theta2 + 2*theta3))/1152921504606846976 + (5575185*d_theta1*d_theta2*sin(2*theta2 - 2*theta5))/89202980794122492566142873090593446023921664 + (5575185*d_theta1*d_theta2*sin(2*theta2 + 2*theta5))/89202980794122492566142873090593446023921664 - (871123*d_theta1*d_theta3*sin(2*theta3 - theta4))/174224571863520493293247799005065324265472 - (d_theta1*d_theta4*sin(2*theta2 - theta4))/2787593149816327892691964784081045188247552 - (d_theta1*d_theta2*sin(2*theta3 - 2*theta5))/89202980794122492566142873090593446023921664 - (d_theta1*d_theta2*sin(2*theta3 + 2*theta5))/89202980794122492566142873090593446023921664 - (d_theta1*d_theta3*sin(2*theta2 - 2*theta5))/89202980794122492566142873090593446023921664 - (d_theta1*d_theta3*sin(2*theta2 + 2*theta5))/89202980794122492566142873090593446023921664 + (61327057*d_theta1*d_theta3*sin(2*theta3 - 2*theta4))/89202980794122492566142873090593446023921664 + (36238715*d_theta1*d_theta3*sin(2*theta3 + 2*theta4))/44601490397061246283071436545296723011960832 + (2854495*d_theta1*d_theta3*sin(2*theta3 - theta5))/5708990770823839524233143877797980545530986496 - (30663525*d_theta1*d_theta4*sin(2*theta2 - 2*theta4))/44601490397061246283071436545296723011960832 + (36238715*d_theta1*d_theta4*sin(2*theta2 + 2*theta4))/44601490397061246283071436545296723011960832 - (d_theta1*d_theta4*sin(2*theta3 - theta4))/2787593149816327892691964784081045188247552 - (d_theta1*d_theta2*sin(2*theta4 - 2*theta5))/89202980794122492566142873090593446023921664 - (d_theta1*d_theta2*sin(2*theta4 + 2*theta5))/89202980794122492566142873090593446023921664 + (5575185*d_theta1*d_theta3*sin(2*theta3 - 2*theta5))/89202980794122492566142873090593446023921664 + (5575185*d_theta1*d_theta3*sin(2*theta3 + 2*theta5))/89202980794122492566142873090593446023921664 - (d_theta1*d_theta4*sin(2*theta2 - 2*theta5))/89202980794122492566142873090593446023921664 - (d_theta1*d_theta4*sin(2*theta2 + 2*theta5))/89202980794122492566142873090593446023921664 - (30663525*d_theta1*d_theta4*sin(2*theta3 - 2*theta4))/44601490397061246283071436545296723011960832 + (36238715*d_theta1*d_theta4*sin(2*theta3 + 2*theta4))/44601490397061246283071436545296723011960832 - (2854495*d_theta1*d_theta5*sin(2*theta2 - theta5))/11417981541647679048466287755595961091061972992 - (d_theta1*d_theta3*sin(2*theta4 - 2*theta5))/89202980794122492566142873090593446023921664 - (d_theta1*d_theta3*sin(2*theta4 + 2*theta5))/89202980794122492566142873090593446023921664 - (d_theta1*d_theta4*sin(2*theta3 - 2*theta5))/89202980794122492566142873090593446023921664 - (d_theta1*d_theta4*sin(2*theta3 + 2*theta5))/89202980794122492566142873090593446023921664 + (2854495*d_theta1*d_theta4*sin(2*theta4 - theta5))/5708990770823839524233143877797980545530986496 - (2787593*d_theta1*d_theta5*sin(2*theta2 - 2*theta5))/44601490397061246283071436545296723011960832 + (5575185*d_theta1*d_theta5*sin(2*theta2 + 2*theta5))/89202980794122492566142873090593446023921664 - (2854495*d_theta1*d_theta5*sin(2*theta3 - theta5))/11417981541647679048466287755595961091061972992 + (5575185*d_theta1*d_theta4*sin(2*theta4 - 2*theta5))/89202980794122492566142873090593446023921664 + (5575185*d_theta1*d_theta4*sin(2*theta4 + 2*theta5))/89202980794122492566142873090593446023921664 - (2787593*d_theta1*d_theta5*sin(2*theta3 - 2*theta5))/44601490397061246283071436545296723011960832 + (5575185*d_theta1*d_theta5*sin(2*theta3 + 2*theta5))/89202980794122492566142873090593446023921664 - (2854495*d_theta1*d_theta5*sin(2*theta4 - theta5))/11417981541647679048466287755595961091061972992 - (2787593*d_theta1*d_theta5*sin(2*theta4 - 2*theta5))/44601490397061246283071436545296723011960832 + (5575185*d_theta1*d_theta5*sin(2*theta4 + 2*theta5))/89202980794122492566142873090593446023921664 + (7988070105025833*d_theta2*d_theta3*cos(theta2 + theta3 - theta5))/4722366482869645213696 + (8313573984755043*d_theta1*d_theta3*cos(theta3 + theta4 - theta5))/18446744073709551616 + (8313573984755043*d_theta1*d_theta4*cos(theta3 + theta4 - theta5))/18446744073709551616 - (8313573984755043*d_theta1*d_theta5*cos(theta3 + theta4 - theta5))/18446744073709551616 - (6968983*d_theta1*d_theta2*sin(theta3 - 2*theta2 + theta4))/696898287454081973172991196020261297061888 - (5387337053181017*d_theta1*d_theta2*sin(2*theta2 + theta3 + theta4))/576460752303423488 - (5387337053181017*d_theta1*d_theta3*sin(2*theta2 + theta3 + theta4))/1152921504606846976 + (21408715*d_theta1*d_theta2*sin(theta4 - 2*theta2 + theta5))/5708990770823839524233143877797980545530986496 - (446015*d_theta1*d_theta2*sin(2*theta2 + theta4 + theta5))/356811923176489970264571492362373784095686656 - (5387337053181017*d_theta1*d_theta4*sin(2*theta2 + theta3 + theta4))/1152921504606846976 - (5571380563941847*d_theta2*d_theta3*sin(theta2 + theta3 - theta5))/9223372036854775808 + (5959870363491779*d_theta1*d_theta3*sin(theta3 + theta4 - theta5))/4722366482869645213696 + (21408715*d_theta1*d_theta3*sin(theta4 - 2*theta3 + theta5))/5708990770823839524233143877797980545530986496 - (446015*d_theta1*d_theta3*sin(2*theta3 + theta4 + theta5))/356811923176489970264571492362373784095686656 + (5959870363491779*d_theta1*d_theta4*sin(theta3 + theta4 - theta5))/4722366482869645213696 + (3568119*d_theta1*d_theta4*sin(2*theta2 + theta4 + theta5))/2854495385411919762116571938898990272765493248 + (3568119*d_theta1*d_theta4*sin(2*theta3 + theta4 + theta5))/2854495385411919762116571938898990272765493248 - (5959870363491779*d_theta1*d_theta5*sin(theta3 + theta4 - theta5))/4722366482869645213696 + (3568119*d_theta1*d_theta5*sin(2*theta2 + theta4 + theta5))/2854495385411919762116571938898990272765493248 + (3568119*d_theta1*d_theta5*sin(2*theta3 + theta4 + theta5))/2854495385411919762116571938898990272765493248 + (9004151162956663*d_theta2*d_theta3*cos(theta2 + theta3 + theta4 + theta5))/18889465931478580854784 + (9004151162956663*d_theta2*d_theta4*cos(theta2 + theta3 + theta4 + theta5))/18889465931478580854784 + (9004151162956663*d_theta3*d_theta4*cos(theta2 + theta3 + theta4 + theta5))/18889465931478580854784 + (4653258611581729*d_theta2*d_theta3*sin(theta2 + theta3 + theta4 + theta5))/36893488147419103232 + (4653258611581729*d_theta2*d_theta4*sin(theta2 + theta3 + theta4 + theta5))/36893488147419103232 + (4653258611581729*d_theta3*d_theta4*sin(theta2 + theta3 + theta4 + theta5))/36893488147419103232 - (8937783066759625*d_theta2*d_theta3*cos(theta2 + theta3))/2305843009213693952 + (5571380563941847*d_theta1*d_theta4*cos(theta4 + theta5))/18446744073709551616 + (5571380563941847*d_theta1*d_theta5*cos(theta4 + theta5))/18446744073709551616 + (5571380563941847*d_theta1*d_theta2*cos(2*theta2 + 2*theta3 + theta4 - theta5))/9223372036854775808 + (22300745*d_theta1*d_theta2*cos(2*theta3 - 2*theta2 + 2*theta4 + theta5))/44601490397061246283071436545296723011960832 + (22300745*d_theta1*d_theta2*cos(2*theta2 - 2*theta3 - 2*theta4 + theta5))/44601490397061246283071436545296723011960832 + (d_theta1*d_theta2*cos(2*theta2 - 2*theta3 + 2*theta4 + theta5))/89202980794122492566142873090593446023921664 + (d_theta1*d_theta2*cos(2*theta2 + 2*theta3 - 2*theta4 + theta5))/89202980794122492566142873090593446023921664 + (4653258611581729*d_theta1*d_theta2*cos(2*theta2 + 2*theta3 + 2*theta4 + theta5))/36893488147419103232 + (5571380563941847*d_theta1*d_theta3*cos(2*theta2 + 2*theta3 + theta4 - theta5))/9223372036854775808 + (d_theta1*d_theta3*cos(2*theta3 - 2*theta2 + 2*theta4 + theta5))/89202980794122492566142873090593446023921664 + (d_theta1*d_theta3*cos(2*theta2 - 2*theta3 - 2*theta4 + theta5))/89202980794122492566142873090593446023921664 + (22300745*d_theta1*d_theta3*cos(2*theta2 - 2*theta3 + 2*theta4 + theta5))/44601490397061246283071436545296723011960832 + (d_theta1*d_theta3*cos(2*theta2 + 2*theta3 - 2*theta4 + theta5))/89202980794122492566142873090593446023921664 + (4653258611581729*d_theta1*d_theta3*cos(2*theta2 + 2*theta3 + 2*theta4 + theta5))/36893488147419103232 + (5571380563941847*d_theta1*d_theta4*cos(2*theta2 + 2*theta3 + theta4 - theta5))/18446744073709551616 + (d_theta1*d_theta4*cos(2*theta3 - 2*theta2 + 2*theta4 + theta5))/89202980794122492566142873090593446023921664 + (d_theta1*d_theta4*cos(2*theta2 - 2*theta3 - 2*theta4 + theta5))/89202980794122492566142873090593446023921664 + (d_theta1*d_theta4*cos(2*theta2 - 2*theta3 + 2*theta4 + theta5))/89202980794122492566142873090593446023921664 + (22300745*d_theta1*d_theta4*cos(2*theta2 + 2*theta3 - 2*theta4 + theta5))/44601490397061246283071436545296723011960832 + (4653258611581729*d_theta1*d_theta4*cos(2*theta2 + 2*theta3 + 2*theta4 + theta5))/36893488147419103232 - (5571380563941847*d_theta1*d_theta5*cos(2*theta2 + 2*theta3 + theta4 - theta5))/18446744073709551616 + (4653258611581729*d_theta1*d_theta5*cos(2*theta2 + 2*theta3 + 2*theta4 + theta5))/73786976294838206464 - (581180430255771*d_theta2*d_theta3*sin(theta2 + theta3))/36028797018963968 - (5387337053181017*d_theta1*d_theta3*sin(theta3 + theta4))/1152921504606846976 - (5387337053181017*d_theta1*d_theta4*sin(theta3 + theta4))/1152921504606846976 - (7988070105025833*d_theta1*d_theta4*sin(theta4 + theta5))/9444732965739290427392 - (7988070105025833*d_theta1*d_theta5*sin(theta4 + theta5))/9444732965739290427392 - (d_theta1*d_theta2*sin(2*theta2 - 2*theta3 + theta4 - theta5))/5708990770823839524233143877797980545530986496 + (7988070105025833*d_theta1*d_theta2*sin(2*theta2 + 2*theta3 + theta4 - theta5))/4722366482869645213696 - (d_theta1*d_theta2*sin(2*theta2 + 2*theta3 - theta4 + theta5))/5708990770823839524233143877797980545530986496 - (9004151162956663*d_theta1*d_theta2*sin(2*theta2 + 2*theta3 + 2*theta4 + theta5))/18889465931478580854784 + (7988070105025833*d_theta1*d_theta3*sin(2*theta2 + 2*theta3 + theta4 - theta5))/4722366482869645213696 - (d_theta1*d_theta3*sin(2*theta2 + 2*theta3 - theta4 + theta5))/5708990770823839524233143877797980545530986496 - (9004151162956663*d_theta1*d_theta3*sin(2*theta2 + 2*theta3 + 2*theta4 + theta5))/18889465931478580854784 + (7988070105025833*d_theta1*d_theta4*sin(2*theta2 + 2*theta3 + theta4 - theta5))/9444732965739290427392 - (9004151162956663*d_theta1*d_theta4*sin(2*theta2 + 2*theta3 + 2*theta4 + theta5))/18889465931478580854784 - (7988070105025833*d_theta1*d_theta5*sin(2*theta2 + 2*theta3 + theta4 - theta5))/9444732965739290427392 - (9004151162956663*d_theta1*d_theta5*sin(2*theta2 + 2*theta3 + 2*theta4 + theta5))/37778931862957161709568;
   (d_theta1^2*sin(theta4))/1393796574908163946345982392040522594123776 - (d_theta1^2*sin(theta5))/5708990770823839524233143877797980545530986496 - (3257081095467945*d_theta3^2*sin(theta3))/288230376151711744 - (7220698343344529*d_theta4^2*sin(theta4))/2305843009213693952 - (9004151162956663*d_theta5^2*sin(theta5))/18889465931478580854784 - (3825825015716409*d_theta1^2*cos(2*theta2))/147573952589676412928 + (4725330594848641*d_theta1^2*sin(2*theta2))/288230376151711744 - (d_theta1^2*cos(theta5))/11150372599265311570767859136324180752990208 - (7028085605816175*d_theta3^2*cos(theta3))/590295810358705651712 + (4653258611581729*d_theta5^2*cos(theta5))/36893488147419103232 - (7028085605816175*d_theta2*d_theta3*cos(theta3))/295147905179352825856 - (3257081095467945*d_theta2*d_theta3*sin(theta3))/144115188075855872 - (7220698343344529*d_theta2*d_theta4*sin(theta4))/1152921504606846976 - (7220698343344529*d_theta3*d_theta4*sin(theta4))/1152921504606846976 + (7028085605816175*d_theta1^2*cos(2*theta2)*cos(theta3))/590295810358705651712 + (3257081095467945*d_theta1^2*cos(2*theta2)*sin(theta3))/288230376151711744 + (3257081095467945*d_theta1^2*sin(2*theta2)*cos(theta3))/288230376151711744 - (13937965*d_theta1^2*cos(2*theta2)*sin(theta4))/2787593149816327892691964784081045188247552 - (13937965*d_theta1^2*sin(2*theta2)*cos(theta4))/2787593149816327892691964784081045188247552 - (2854495*d_theta1^2*cos(2*theta2)*sin(theta5))/5708990770823839524233143877797980545530986496 - (7028085605816175*d_theta1^2*sin(2*theta2)*sin(theta3))/590295810358705651712 - (2282168433090971*d_theta2*d_theta5*cos(2*theta5))/9444732965739290427392 - (2282168433090971*d_theta3*d_theta5*cos(2*theta5))/9444732965739290427392 - (2282168433090971*d_theta4*d_theta5*cos(2*theta5))/9444732965739290427392 - (3240011242931075*d_theta2*d_theta5*sin(2*theta5))/18446744073709551616 - (3240011242931075*d_theta3*d_theta5*sin(2*theta5))/18446744073709551616 - (3240011242931075*d_theta4*d_theta5*sin(2*theta5))/18446744073709551616 + (1007824040173657*d_theta1^2*cos(2*theta2)*cos(2*theta3))/288230376151711744 - (d_theta1^2*cos(2*theta2)*cos(2*theta5))/91343852333181432387730302044767688728495783936 - (8356542075167085*d_theta1^2*cos(2*theta2)*sin(2*theta3))/2305843009213693952 - (8356542075167085*d_theta1^2*cos(2*theta3)*sin(2*theta2))/2305843009213693952 + (2787593*d_theta1^2*cos(2*theta2)*sin(2*theta4))/5575186299632655785383929568162090376495104 - (1393797*d_theta1^2*cos(2*theta4)*sin(2*theta2))/22300745198530623141535718272648361505980416 - (1393797*d_theta1^2*cos(2*theta5)*sin(2*theta2))/22300745198530623141535718272648361505980416 - (1007824040173657*d_theta1^2*sin(2*theta2)*sin(2*theta3))/288230376151711744 - (17126969*d_theta1^2*sin(2*theta2)*sin(2*theta5))/91343852333181432387730302044767688728495783936 + (5571380563941847*d_theta4^2*cos(theta4)*cos(theta5))/9223372036854775808 + (5571380563941847*d_theta5^2*cos(theta4)*cos(theta5))/9223372036854775808 - (5387337053181017*d_theta3^2*cos(theta3)*sin(theta4))/1152921504606846976 - (5387337053181017*d_theta3^2*cos(theta4)*sin(theta3))/1152921504606846976 - (5387337053181017*d_theta4^2*cos(theta3)*sin(theta4))/1152921504606846976 - (5387337053181017*d_theta4^2*cos(theta4)*sin(theta3))/1152921504606846976 - (7988070105025833*d_theta4^2*cos(theta4)*sin(theta5))/4722366482869645213696 - (7988070105025833*d_theta5^2*cos(theta4)*sin(theta5))/4722366482869645213696 + (5387337053181017*d_theta1^2*cos(2*theta2)*cos(theta3)*sin(theta4))/1152921504606846976 + (5387337053181017*d_theta1^2*cos(2*theta2)*cos(theta4)*sin(theta3))/1152921504606846976 + (5387337053181017*d_theta1^2*sin(2*theta2)*cos(theta3)*cos(theta4))/1152921504606846976 - (5387337053181017*d_theta1^2*sin(2*theta2)*sin(theta3)*sin(theta4))/1152921504606846976 + (3568119*d_theta1^2*sin(2*theta2)*sin(theta4)*sin(theta5))/1427247692705959881058285969449495136382746624 + (7220698343344529*d_theta1^2*cos(2*theta2)*cos(2*theta3)*sin(theta4))/2305843009213693952 + (7220698343344529*d_theta1^2*cos(2*theta2)*sin(2*theta3)*cos(theta4))/2305843009213693952 + (7220698343344529*d_theta1^2*cos(2*theta3)*sin(2*theta2)*cos(theta4))/2305843009213693952 - (2854495*d_theta1^2*cos(2*theta2)*cos(2*theta3)*sin(theta5))/5708990770823839524233143877797980545530986496 - (2854495*d_theta1^2*cos(2*theta2)*cos(2*theta4)*sin(theta5))/5708990770823839524233143877797980545530986496 + (2787593*d_theta1^2*sin(2*theta2)*sin(2*theta3)*cos(theta5))/5575186299632655785383929568162090376495104 + (2787593*d_theta1^2*sin(2*theta2)*sin(2*theta4)*cos(theta5))/5575186299632655785383929568162090376495104 - (7220698343344529*d_theta1^2*sin(2*theta2)*sin(2*theta3)*sin(theta4))/2305843009213693952 + (8313573984755043*d_theta3^2*cos(theta3)*cos(theta4)*cos(theta5))/9223372036854775808 + (8313573984755043*d_theta4^2*cos(theta3)*cos(theta4)*cos(theta5))/9223372036854775808 + (8313573984755043*d_theta5^2*cos(theta3)*cos(theta4)*cos(theta5))/9223372036854775808 - (5959870363491779*d_theta3^2*cos(theta3)*cos(theta4)*sin(theta5))/2361183241434822606848 - (5959870363491779*d_theta4^2*cos(theta3)*cos(theta4)*sin(theta5))/2361183241434822606848 - (5959870363491779*d_theta5^2*cos(theta3)*cos(theta4)*sin(theta5))/2361183241434822606848 + (2695991646372651*d_theta1^2*cos(2*theta2)*cos(2*theta3)*cos(2*theta4))/9223372036854775808 - (8313573984755043*d_theta3^2*cos(theta5)*sin(theta3)*sin(theta4))/9223372036854775808 - (8313573984755043*d_theta4^2*cos(theta5)*sin(theta3)*sin(theta4))/9223372036854775808 - (8313573984755043*d_theta5^2*cos(theta5)*sin(theta3)*sin(theta4))/9223372036854775808 + (5571380563941847*d_theta2*d_theta4*cos(theta4)*cos(theta5))/4611686018427387904 + (5571380563941847*d_theta3*d_theta4*cos(theta4)*cos(theta5))/4611686018427387904 + (1160499590055099*d_theta1^2*cos(2*theta2)*cos(2*theta3)*sin(2*theta4))/4611686018427387904 + (1160499590055099*d_theta1^2*cos(2*theta2)*cos(2*theta4)*sin(2*theta3))/4611686018427387904 + (1160499590055099*d_theta1^2*cos(2*theta3)*cos(2*theta4)*sin(2*theta2))/4611686018427387904 - (d_theta1^2*cos(2*theta2)*cos(2*theta3)*sin(2*theta5))/356811923176489970264571492362373784095686656 - (d_theta1^2*cos(2*theta2)*cos(2*theta5)*sin(2*theta3))/356811923176489970264571492362373784095686656 - (22300751*d_theta1^2*cos(2*theta3)*cos(2*theta5)*sin(2*theta2))/356811923176489970264571492362373784095686656 - (d_theta1^2*cos(2*theta2)*cos(2*theta4)*sin(2*theta5))/356811923176489970264571492362373784095686656 - (d_theta1^2*cos(2*theta2)*cos(2*theta5)*sin(2*theta4))/356811923176489970264571492362373784095686656 - (22300751*d_theta1^2*cos(2*theta4)*cos(2*theta5)*sin(2*theta2))/356811923176489970264571492362373784095686656 + (5959870363491779*d_theta3^2*sin(theta3)*sin(theta4)*sin(theta5))/2361183241434822606848 + (5959870363491779*d_theta4^2*sin(theta3)*sin(theta4)*sin(theta5))/2361183241434822606848 + (5959870363491779*d_theta5^2*sin(theta3)*sin(theta4)*sin(theta5))/2361183241434822606848 - (5387337053181017*d_theta2*d_theta3*cos(theta3)*sin(theta4))/576460752303423488 - (5387337053181017*d_theta2*d_theta3*cos(theta4)*sin(theta3))/576460752303423488 + (8313573984755043*d_theta1*d_theta5*cos(theta5)*sin(theta2))/4611686018427387904 - (5387337053181017*d_theta2*d_theta4*cos(theta3)*sin(theta4))/576460752303423488 - (5387337053181017*d_theta2*d_theta4*cos(theta4)*sin(theta3))/576460752303423488 - (5387337053181017*d_theta3*d_theta4*cos(theta3)*sin(theta4))/576460752303423488 - (5387337053181017*d_theta3*d_theta4*cos(theta4)*sin(theta3))/576460752303423488 - (7988070105025833*d_theta2*d_theta4*cos(theta4)*sin(theta5))/2361183241434822606848 - (7988070105025833*d_theta2*d_theta5*cos(theta5)*sin(theta4))/2361183241434822606848 - (7988070105025833*d_theta3*d_theta4*cos(theta4)*sin(theta5))/2361183241434822606848 - (7988070105025833*d_theta3*d_theta5*cos(theta5)*sin(theta4))/2361183241434822606848 - (7988070105025833*d_theta4*d_theta5*cos(theta5)*sin(theta4))/2361183241434822606848 - (2695991646372651*d_theta1^2*cos(2*theta2)*sin(2*theta3)*sin(2*theta4))/9223372036854775808 - (2695991646372651*d_theta1^2*cos(2*theta3)*sin(2*theta2)*sin(2*theta4))/9223372036854775808 - (2695991646372651*d_theta1^2*cos(2*theta4)*sin(2*theta2)*sin(2*theta3))/9223372036854775808 + (11417979*d_theta1^2*cos(2*theta2)*sin(2*theta3)*sin(2*theta5))/91343852333181432387730302044767688728495783936 - (2854495*d_theta1^2*cos(2*theta3)*sin(2*theta2)*sin(2*theta5))/45671926166590716193865151022383844364247891968 - (d_theta1^2*cos(2*theta5)*sin(2*theta2)*sin(2*theta3))/91343852333181432387730302044767688728495783936 + (11417979*d_theta1^2*cos(2*theta2)*sin(2*theta4)*sin(2*theta5))/91343852333181432387730302044767688728495783936 - (2854495*d_theta1^2*cos(2*theta4)*sin(2*theta2)*sin(2*theta5))/45671926166590716193865151022383844364247891968 - (d_theta1^2*cos(2*theta5)*sin(2*theta2)*sin(2*theta4))/91343852333181432387730302044767688728495783936 - (5959870363491779*d_theta1*d_theta5*sin(theta2)*sin(theta5))/1180591620717411303424 - (5571380563941847*d_theta2*d_theta5*sin(theta4)*sin(theta5))/4611686018427387904 - (5571380563941847*d_theta3*d_theta5*sin(theta4)*sin(theta5))/4611686018427387904 - (5571380563941847*d_theta4*d_theta5*sin(theta4)*sin(theta5))/4611686018427387904 - (1160499590055099*d_theta1^2*sin(2*theta2)*sin(2*theta3)*sin(2*theta4))/4611686018427387904 - (d_theta1^2*sin(2*theta2)*sin(2*theta3)*sin(2*theta5))/356811923176489970264571492362373784095686656 - (d_theta1^2*sin(2*theta2)*sin(2*theta4)*sin(2*theta5))/356811923176489970264571492362373784095686656 + (10050494243446848990263944093682850882789*d_theta1^2*cos(2*theta2)*cos(theta5)*sin(theta3)*sin(theta4))/11150372599265311570767859136324180752990208 + (10050494243446848990263944093682862033161*d_theta1^2*sin(2*theta2)*cos(theta3)*cos(theta5)*sin(theta4))/11150372599265311570767859136324180752990208 + (10050494243446848990263944093682862033161*d_theta1^2*sin(2*theta2)*cos(theta4)*cos(theta5)*sin(theta3))/11150372599265311570767859136324180752990208 - (3240011242931075*d_theta1^2*cos(2*theta2)*cos(2*theta3)*cos(2*theta5)*sin(2*theta4))/73786976294838206464 - (3240011242931075*d_theta1^2*cos(2*theta2)*cos(2*theta4)*cos(2*theta5)*sin(2*theta3))/73786976294838206464 - (3240011242931075*d_theta1^2*cos(2*theta3)*cos(2*theta4)*cos(2*theta5)*sin(2*theta2))/73786976294838206464 - (5959870363491779*d_theta1^2*cos(2*theta2)*sin(theta3)*sin(theta4)*sin(theta5))/2361183241434822606848 - (5959870363491779*d_theta1^2*sin(2*theta2)*cos(theta3)*sin(theta4)*sin(theta5))/2361183241434822606848 - (5959870363491779*d_theta1^2*sin(2*theta2)*cos(theta4)*sin(theta3)*sin(theta5))/2361183241434822606848 + (2282168433090971*d_theta1^2*cos(2*theta2)*cos(2*theta3)*sin(2*theta4)*sin(2*theta5))/37778931862957161709568 + (2282168433090971*d_theta1^2*cos(2*theta2)*cos(2*theta4)*sin(2*theta3)*sin(2*theta5))/37778931862957161709568 + (2282168433090971*d_theta1^2*cos(2*theta3)*cos(2*theta4)*sin(2*theta2)*sin(2*theta5))/37778931862957161709568 + (3240011242931075*d_theta1^2*cos(2*theta5)*sin(2*theta2)*sin(2*theta3)*sin(2*theta4))/73786976294838206464 - (2282168433090971*d_theta1^2*sin(2*theta2)*sin(2*theta3)*sin(2*theta4)*sin(2*theta5))/37778931862957161709568 - (5571380563941847*d_theta1^2*cos(2*theta2)*cos(2*theta3)*cos(theta4)*cos(theta5))/9223372036854775808 + (7988070105025833*d_theta1^2*cos(2*theta2)*cos(2*theta3)*cos(theta4)*sin(theta5))/4722366482869645213696 + (5571380563941847*d_theta1^2*cos(2*theta2)*sin(2*theta3)*cos(theta5)*sin(theta4))/9223372036854775808 + (5571380563941847*d_theta1^2*cos(2*theta3)*sin(2*theta2)*cos(theta5)*sin(theta4))/9223372036854775808 + (5571380563941847*d_theta1^2*sin(2*theta2)*sin(2*theta3)*cos(theta4)*cos(theta5))/9223372036854775808 - (7988070105025833*d_theta1^2*cos(2*theta2)*sin(2*theta3)*sin(theta4)*sin(theta5))/4722366482869645213696 - (7988070105025833*d_theta1^2*cos(2*theta3)*sin(2*theta2)*sin(theta4)*sin(theta5))/4722366482869645213696 - (7988070105025833*d_theta1^2*sin(2*theta2)*sin(2*theta3)*cos(theta4)*sin(theta5))/4722366482869645213696 - (4653258611581729*d_theta1^2*cos(2*theta2)*cos(2*theta3)*cos(2*theta4)*cos(theta5))/36893488147419103232 - (1951319518623669*d_theta1*d_theta5*cos(theta2)*cos(theta3)*cos(theta4))/9223372036854775808 + (8313573984755043*d_theta2*d_theta3*cos(theta3)*cos(theta4)*cos(theta5))/4611686018427387904 + (8313573984755043*d_theta2*d_theta4*cos(theta3)*cos(theta4)*cos(theta5))/4611686018427387904 + (8313573984755043*d_theta3*d_theta4*cos(theta3)*cos(theta4)*cos(theta5))/4611686018427387904 + (9004151162956663*d_theta1^2*cos(2*theta2)*cos(2*theta3)*cos(2*theta4)*sin(theta5))/18889465931478580854784 + (5571380563941847*d_theta1*d_theta5*cos(theta2)*cos(theta5)*sin(theta3))/4611686018427387904 + (5571380563941847*d_theta1*d_theta5*cos(theta3)*cos(theta5)*sin(theta2))/4611686018427387904 - (5959870363491779*d_theta2*d_theta3*cos(theta3)*cos(theta4)*sin(theta5))/1180591620717411303424 - (5959870363491779*d_theta2*d_theta4*cos(theta3)*cos(theta4)*sin(theta5))/1180591620717411303424 - (5959870363491779*d_theta2*d_theta5*cos(theta3)*cos(theta5)*sin(theta4))/1180591620717411303424 - (5959870363491779*d_theta2*d_theta5*cos(theta4)*cos(theta5)*sin(theta3))/1180591620717411303424 - (5959870363491779*d_theta3*d_theta4*cos(theta3)*cos(theta4)*sin(theta5))/1180591620717411303424 - (5959870363491779*d_theta3*d_theta5*cos(theta3)*cos(theta5)*sin(theta4))/1180591620717411303424 - (5959870363491779*d_theta3*d_theta5*cos(theta4)*cos(theta5)*sin(theta3))/1180591620717411303424 - (5959870363491779*d_theta4*d_theta5*cos(theta3)*cos(theta5)*sin(theta4))/1180591620717411303424 - (5959870363491779*d_theta4*d_theta5*cos(theta4)*cos(theta5)*sin(theta3))/1180591620717411303424 + (4653258611581729*d_theta1^2*cos(2*theta2)*sin(2*theta3)*sin(2*theta4)*cos(theta5))/36893488147419103232 + (4653258611581729*d_theta1^2*cos(2*theta3)*sin(2*theta2)*sin(2*theta4)*cos(theta5))/36893488147419103232 + (4653258611581729*d_theta1^2*cos(2*theta4)*sin(2*theta2)*sin(2*theta3)*cos(theta5))/36893488147419103232 + (1951319518623669*d_theta1*d_theta5*cos(theta2)*sin(theta3)*sin(theta4))/9223372036854775808 + (1951319518623669*d_theta1*d_theta5*cos(theta3)*sin(theta2)*sin(theta4))/9223372036854775808 + (1951319518623669*d_theta1*d_theta5*cos(theta4)*sin(theta2)*sin(theta3))/9223372036854775808 - (7988070105025833*d_theta1*d_theta5*cos(theta2)*sin(theta3)*sin(theta5))/2361183241434822606848 - (7988070105025833*d_theta1*d_theta5*cos(theta3)*sin(theta2)*sin(theta5))/2361183241434822606848 - (8313573984755043*d_theta2*d_theta3*cos(theta5)*sin(theta3)*sin(theta4))/4611686018427387904 - (8313573984755043*d_theta2*d_theta4*cos(theta5)*sin(theta3)*sin(theta4))/4611686018427387904 - (8313573984755043*d_theta2*d_theta5*cos(theta3)*sin(theta4)*sin(theta5))/4611686018427387904 - (8313573984755043*d_theta2*d_theta5*cos(theta4)*sin(theta3)*sin(theta5))/4611686018427387904 - (8313573984755043*d_theta3*d_theta4*cos(theta5)*sin(theta3)*sin(theta4))/4611686018427387904 - (8313573984755043*d_theta3*d_theta5*cos(theta3)*sin(theta4)*sin(theta5))/4611686018427387904 - (8313573984755043*d_theta3*d_theta5*cos(theta4)*sin(theta3)*sin(theta5))/4611686018427387904 - (8313573984755043*d_theta4*d_theta5*cos(theta3)*sin(theta4)*sin(theta5))/4611686018427387904 - (8313573984755043*d_theta4*d_theta5*cos(theta4)*sin(theta3)*sin(theta5))/4611686018427387904 - (9004151162956663*d_theta1^2*cos(2*theta2)*sin(2*theta3)*sin(2*theta4)*sin(theta5))/18889465931478580854784 - (9004151162956663*d_theta1^2*cos(2*theta3)*sin(2*theta2)*sin(2*theta4)*sin(theta5))/18889465931478580854784 - (9004151162956663*d_theta1^2*cos(2*theta4)*sin(2*theta2)*sin(2*theta3)*sin(theta5))/18889465931478580854784 + (5959870363491779*d_theta2*d_theta3*sin(theta3)*sin(theta4)*sin(theta5))/1180591620717411303424 + (5959870363491779*d_theta2*d_theta4*sin(theta3)*sin(theta4)*sin(theta5))/1180591620717411303424 + (5959870363491779*d_theta3*d_theta4*sin(theta3)*sin(theta4)*sin(theta5))/1180591620717411303424 - (10050494243446848990263944093682862033161*d_theta1^2*cos(2*theta2)*cos(theta3)*cos(theta4)*cos(theta5))/11150372599265311570767859136324180752990208 + (5959870363491779*d_theta1^2*cos(2*theta2)*cos(theta3)*cos(theta4)*sin(theta5))/2361183241434822606848 + (3240011242931075*d_theta1*d_theta5*cos(2*theta5)*cos(theta2)*sin(theta3)*sin(theta4))/18446744073709551616 + (3240011242931075*d_theta1*d_theta5*cos(2*theta5)*cos(theta3)*sin(theta2)*sin(theta4))/18446744073709551616 + (3240011242931075*d_theta1*d_theta5*cos(2*theta5)*cos(theta4)*sin(theta2)*sin(theta3))/18446744073709551616 - (2282168433090971*d_theta1*d_theta5*sin(2*theta5)*cos(theta2)*sin(theta3)*sin(theta4))/9444732965739290427392 - (2282168433090971*d_theta1*d_theta5*sin(2*theta5)*cos(theta3)*sin(theta2)*sin(theta4))/9444732965739290427392 - (2282168433090971*d_theta1*d_theta5*sin(2*theta5)*cos(theta4)*sin(theta2)*sin(theta3))/9444732965739290427392 + (4653258611581729*d_theta1*d_theta5*cos(theta2)*cos(theta3)*cos(theta5)*sin(theta4))/18446744073709551616 + (4653258611581729*d_theta1*d_theta5*cos(theta2)*cos(theta4)*cos(theta5)*sin(theta3))/18446744073709551616 + (4653258611581729*d_theta1*d_theta5*cos(theta3)*cos(theta4)*cos(theta5)*sin(theta2))/18446744073709551616 - (9004151162956663*d_theta1*d_theta5*cos(theta2)*cos(theta3)*sin(theta4)*sin(theta5))/9444732965739290427392 - (9004151162956663*d_theta1*d_theta5*cos(theta2)*cos(theta4)*sin(theta3)*sin(theta5))/9444732965739290427392 - (9004151162956663*d_theta1*d_theta5*cos(theta3)*cos(theta4)*sin(theta2)*sin(theta5))/9444732965739290427392 - (4653258611581729*d_theta1*d_theta5*cos(theta5)*sin(theta2)*sin(theta3)*sin(theta4))/18446744073709551616 + (9004151162956663*d_theta1*d_theta5*sin(theta2)*sin(theta3)*sin(theta4)*sin(theta5))/9444732965739290427392 - (3240011242931075*d_theta1*d_theta5*cos(2*theta5)*cos(theta2)*cos(theta3)*cos(theta4))/18446744073709551616 + (2282168433090971*d_theta1*d_theta5*sin(2*theta5)*cos(theta2)*cos(theta3)*cos(theta4))/9444732965739290427392;
   (3257081095467945*d_theta1^2*sin(theta3))/576460752303423488 + (d_theta1^2*sin(theta4))/1393796574908163946345982392040522594123776 + (3257081095467945*d_theta2^2*sin(theta3))/288230376151711744 - (d_theta1^2*sin(theta5))/5708990770823839524233143877797980545530986496 - (7220698343344529*d_theta4^2*sin(theta4))/2305843009213693952 - (9004151162956663*d_theta5^2*sin(theta5))/18889465931478580854784 - (1393797*d_theta1^2*sin(2*theta3))/22300745198530623141535718272648361505980416 + (7028085605816175*d_theta1^2*cos(theta3))/1180591620717411303424 + (7028085605816175*d_theta2^2*cos(theta3))/590295810358705651712 - (d_theta1^2*cos(theta5))/11150372599265311570767859136324180752990208 + (4653258611581729*d_theta5^2*cos(theta5))/36893488147419103232 - (7220698343344529*d_theta2*d_theta4*sin(theta4))/1152921504606846976 - (7220698343344529*d_theta3*d_theta4*sin(theta4))/1152921504606846976 + (7028085605816175*d_theta1^2*cos(2*theta2)*cos(theta3))/1180591620717411303424 + (3257081095467945*d_theta1^2*cos(2*theta2)*sin(theta3))/576460752303423488 + (3257081095467945*d_theta1^2*sin(2*theta2)*cos(theta3))/576460752303423488 - (13937965*d_theta1^2*cos(2*theta3)*sin(theta4))/2787593149816327892691964784081045188247552 - (13937965*d_theta1^2*sin(2*theta3)*cos(theta4))/2787593149816327892691964784081045188247552 - (2854495*d_theta1^2*cos(2*theta3)*sin(theta5))/5708990770823839524233143877797980545530986496 - (7028085605816175*d_theta1^2*sin(2*theta2)*sin(theta3))/1180591620717411303424 - (2282168433090971*d_theta2*d_theta5*cos(2*theta5))/9444732965739290427392 - (2282168433090971*d_theta3*d_theta5*cos(2*theta5))/9444732965739290427392 - (2282168433090971*d_theta4*d_theta5*cos(2*theta5))/9444732965739290427392 - (3240011242931075*d_theta2*d_theta5*sin(2*theta5))/18446744073709551616 - (3240011242931075*d_theta3*d_theta5*sin(2*theta5))/18446744073709551616 - (3240011242931075*d_theta4*d_theta5*sin(2*theta5))/18446744073709551616 + (1007824040173657*d_theta1^2*cos(2*theta2)*cos(2*theta3))/288230376151711744 - (d_theta1^2*cos(2*theta3)*cos(2*theta5))/91343852333181432387730302044767688728495783936 - (8356542075167085*d_theta1^2*cos(2*theta2)*sin(2*theta3))/2305843009213693952 - (8356542075167085*d_theta1^2*cos(2*theta3)*sin(2*theta2))/2305843009213693952 + (2787593*d_theta1^2*cos(2*theta3)*sin(2*theta4))/5575186299632655785383929568162090376495104 - (1393797*d_theta1^2*cos(2*theta4)*sin(2*theta3))/22300745198530623141535718272648361505980416 - (1393797*d_theta1^2*cos(2*theta5)*sin(2*theta3))/22300745198530623141535718272648361505980416 - (1007824040173657*d_theta1^2*sin(2*theta2)*sin(2*theta3))/288230376151711744 - (17126969*d_theta1^2*sin(2*theta3)*sin(2*theta5))/91343852333181432387730302044767688728495783936 + (5571380563941847*d_theta4^2*cos(theta4)*cos(theta5))/9223372036854775808 + (5571380563941847*d_theta5^2*cos(theta4)*cos(theta5))/9223372036854775808 + (5387337053181017*d_theta1^2*cos(theta3)*sin(theta4))/2305843009213693952 + (5387337053181017*d_theta1^2*cos(theta4)*sin(theta3))/2305843009213693952 + (5387337053181017*d_theta2^2*cos(theta3)*sin(theta4))/1152921504606846976 + (5387337053181017*d_theta2^2*cos(theta4)*sin(theta3))/1152921504606846976 - (7988070105025833*d_theta4^2*cos(theta4)*sin(theta5))/4722366482869645213696 - (7988070105025833*d_theta5^2*cos(theta4)*sin(theta5))/4722366482869645213696 + (5387337053181017*d_theta1^2*cos(2*theta2)*cos(theta3)*sin(theta4))/2305843009213693952 + (5387337053181017*d_theta1^2*cos(2*theta2)*cos(theta4)*sin(theta3))/2305843009213693952 + (5387337053181017*d_theta1^2*sin(2*theta2)*cos(theta3)*cos(theta4))/2305843009213693952 - (5387337053181017*d_theta1^2*sin(2*theta2)*sin(theta3)*sin(theta4))/2305843009213693952 + (3568119*d_theta1^2*sin(2*theta3)*sin(theta4)*sin(theta5))/1427247692705959881058285969449495136382746624 + (7220698343344529*d_theta1^2*cos(2*theta2)*cos(2*theta3)*sin(theta4))/2305843009213693952 + (7220698343344529*d_theta1^2*cos(2*theta2)*sin(2*theta3)*cos(theta4))/2305843009213693952 + (7220698343344529*d_theta1^2*cos(2*theta3)*sin(2*theta2)*cos(theta4))/2305843009213693952 - (2854495*d_theta1^2*cos(2*theta2)*cos(2*theta3)*sin(theta5))/5708990770823839524233143877797980545530986496 - (2854495*d_theta1^2*cos(2*theta3)*cos(2*theta4)*sin(theta5))/5708990770823839524233143877797980545530986496 + (2787593*d_theta1^2*sin(2*theta2)*sin(2*theta3)*cos(theta5))/5575186299632655785383929568162090376495104 + (2787593*d_theta1^2*sin(2*theta3)*sin(2*theta4)*cos(theta5))/5575186299632655785383929568162090376495104 - (7220698343344529*d_theta1^2*sin(2*theta2)*sin(2*theta3)*sin(theta4))/2305843009213693952 - (8313573984755043*d_theta1^2*cos(theta3)*cos(theta4)*cos(theta5))/18446744073709551616 - (8313573984755043*d_theta2^2*cos(theta3)*cos(theta4)*cos(theta5))/9223372036854775808 + (5959870363491779*d_theta1^2*cos(theta3)*cos(theta4)*sin(theta5))/4722366482869645213696 + (5959870363491779*d_theta2^2*cos(theta3)*cos(theta4)*sin(theta5))/2361183241434822606848 + (2695991646372651*d_theta1^2*cos(2*theta2)*cos(2*theta3)*cos(2*theta4))/9223372036854775808 + (8313573984755043*d_theta1^2*cos(theta5)*sin(theta3)*sin(theta4))/18446744073709551616 + (8313573984755043*d_theta2^2*cos(theta5)*sin(theta3)*sin(theta4))/9223372036854775808 + (5571380563941847*d_theta2*d_theta4*cos(theta4)*cos(theta5))/4611686018427387904 + (5571380563941847*d_theta3*d_theta4*cos(theta4)*cos(theta5))/4611686018427387904 + (1160499590055099*d_theta1^2*cos(2*theta2)*cos(2*theta3)*sin(2*theta4))/4611686018427387904 + (1160499590055099*d_theta1^2*cos(2*theta2)*cos(2*theta4)*sin(2*theta3))/4611686018427387904 + (1160499590055099*d_theta1^2*cos(2*theta3)*cos(2*theta4)*sin(2*theta2))/4611686018427387904 - (d_theta1^2*cos(2*theta2)*cos(2*theta3)*sin(2*theta5))/356811923176489970264571492362373784095686656 - (22300751*d_theta1^2*cos(2*theta2)*cos(2*theta5)*sin(2*theta3))/356811923176489970264571492362373784095686656 - (d_theta1^2*cos(2*theta3)*cos(2*theta5)*sin(2*theta2))/356811923176489970264571492362373784095686656 - (d_theta1^2*cos(2*theta3)*cos(2*theta4)*sin(2*theta5))/356811923176489970264571492362373784095686656 - (d_theta1^2*cos(2*theta3)*cos(2*theta5)*sin(2*theta4))/356811923176489970264571492362373784095686656 - (22300751*d_theta1^2*cos(2*theta4)*cos(2*theta5)*sin(2*theta3))/356811923176489970264571492362373784095686656 - (5959870363491779*d_theta1^2*sin(theta3)*sin(theta4)*sin(theta5))/4722366482869645213696 - (5959870363491779*d_theta2^2*sin(theta3)*sin(theta4)*sin(theta5))/2361183241434822606848 - (7988070105025833*d_theta2*d_theta4*cos(theta4)*sin(theta5))/2361183241434822606848 - (7988070105025833*d_theta2*d_theta5*cos(theta5)*sin(theta4))/2361183241434822606848 - (7988070105025833*d_theta3*d_theta4*cos(theta4)*sin(theta5))/2361183241434822606848 - (7988070105025833*d_theta3*d_theta5*cos(theta5)*sin(theta4))/2361183241434822606848 - (7988070105025833*d_theta4*d_theta5*cos(theta5)*sin(theta4))/2361183241434822606848 - (2695991646372651*d_theta1^2*cos(2*theta2)*sin(2*theta3)*sin(2*theta4))/9223372036854775808 - (2695991646372651*d_theta1^2*cos(2*theta3)*sin(2*theta2)*sin(2*theta4))/9223372036854775808 - (2695991646372651*d_theta1^2*cos(2*theta4)*sin(2*theta2)*sin(2*theta3))/9223372036854775808 - (2854495*d_theta1^2*cos(2*theta2)*sin(2*theta3)*sin(2*theta5))/45671926166590716193865151022383844364247891968 + (11417979*d_theta1^2*cos(2*theta3)*sin(2*theta2)*sin(2*theta5))/91343852333181432387730302044767688728495783936 - (d_theta1^2*cos(2*theta5)*sin(2*theta2)*sin(2*theta3))/91343852333181432387730302044767688728495783936 + (11417979*d_theta1^2*cos(2*theta3)*sin(2*theta4)*sin(2*theta5))/91343852333181432387730302044767688728495783936 - (2854495*d_theta1^2*cos(2*theta4)*sin(2*theta3)*sin(2*theta5))/45671926166590716193865151022383844364247891968 - (d_theta1^2*cos(2*theta5)*sin(2*theta3)*sin(2*theta4))/91343852333181432387730302044767688728495783936 - (5571380563941847*d_theta2*d_theta5*sin(theta4)*sin(theta5))/4611686018427387904 - (5571380563941847*d_theta3*d_theta5*sin(theta4)*sin(theta5))/4611686018427387904 - (5571380563941847*d_theta4*d_theta5*sin(theta4)*sin(theta5))/4611686018427387904 - (1160499590055099*d_theta1^2*sin(2*theta2)*sin(2*theta3)*sin(2*theta4))/4611686018427387904 - (d_theta1^2*sin(2*theta2)*sin(2*theta3)*sin(2*theta5))/356811923176489970264571492362373784095686656 - (d_theta1^2*sin(2*theta3)*sin(2*theta4)*sin(2*theta5))/356811923176489970264571492362373784095686656 + (8313573984755043*d_theta1^2*cos(2*theta2)*cos(theta5)*sin(theta3)*sin(theta4))/18446744073709551616 + (8313573984755043*d_theta1^2*sin(2*theta2)*cos(theta3)*cos(theta5)*sin(theta4))/18446744073709551616 + (8313573984755043*d_theta1^2*sin(2*theta2)*cos(theta4)*cos(theta5)*sin(theta3))/18446744073709551616 - (3240011242931075*d_theta1^2*cos(2*theta2)*cos(2*theta3)*cos(2*theta5)*sin(2*theta4))/73786976294838206464 - (3240011242931075*d_theta1^2*cos(2*theta2)*cos(2*theta4)*cos(2*theta5)*sin(2*theta3))/73786976294838206464 - (3240011242931075*d_theta1^2*cos(2*theta3)*cos(2*theta4)*cos(2*theta5)*sin(2*theta2))/73786976294838206464 - (5959870363491779*d_theta1^2*cos(2*theta2)*sin(theta3)*sin(theta4)*sin(theta5))/4722366482869645213696 - (5959870363491779*d_theta1^2*sin(2*theta2)*cos(theta3)*sin(theta4)*sin(theta5))/4722366482869645213696 - (5959870363491779*d_theta1^2*sin(2*theta2)*cos(theta4)*sin(theta3)*sin(theta5))/4722366482869645213696 + (2282168433090971*d_theta1^2*cos(2*theta2)*cos(2*theta3)*sin(2*theta4)*sin(2*theta5))/37778931862957161709568 + (2282168433090971*d_theta1^2*cos(2*theta2)*cos(2*theta4)*sin(2*theta3)*sin(2*theta5))/37778931862957161709568 + (2282168433090971*d_theta1^2*cos(2*theta3)*cos(2*theta4)*sin(2*theta2)*sin(2*theta5))/37778931862957161709568 + (3240011242931075*d_theta1^2*cos(2*theta5)*sin(2*theta2)*sin(2*theta3)*sin(2*theta4))/73786976294838206464 - (2282168433090971*d_theta1^2*sin(2*theta2)*sin(2*theta3)*sin(2*theta4)*sin(2*theta5))/37778931862957161709568 - (5571380563941847*d_theta1^2*cos(2*theta2)*cos(2*theta3)*cos(theta4)*cos(theta5))/9223372036854775808 + (7988070105025833*d_theta1^2*cos(2*theta2)*cos(2*theta3)*cos(theta4)*sin(theta5))/4722366482869645213696 + (5571380563941847*d_theta1^2*cos(2*theta2)*sin(2*theta3)*cos(theta5)*sin(theta4))/9223372036854775808 + (5571380563941847*d_theta1^2*cos(2*theta3)*sin(2*theta2)*cos(theta5)*sin(theta4))/9223372036854775808 + (5571380563941847*d_theta1^2*sin(2*theta2)*sin(2*theta3)*cos(theta4)*cos(theta5))/9223372036854775808 - (7988070105025833*d_theta1^2*cos(2*theta2)*sin(2*theta3)*sin(theta4)*sin(theta5))/4722366482869645213696 - (7988070105025833*d_theta1^2*cos(2*theta3)*sin(2*theta2)*sin(theta4)*sin(theta5))/4722366482869645213696 - (7988070105025833*d_theta1^2*sin(2*theta2)*sin(2*theta3)*cos(theta4)*sin(theta5))/4722366482869645213696 - (4653258611581729*d_theta1^2*cos(2*theta2)*cos(2*theta3)*cos(2*theta4)*cos(theta5))/36893488147419103232 - (1951319518623669*d_theta1*d_theta5*cos(theta2)*cos(theta3)*cos(theta4))/9223372036854775808 + (9004151162956663*d_theta1^2*cos(2*theta2)*cos(2*theta3)*cos(2*theta4)*sin(theta5))/18889465931478580854784 + (5571380563941847*d_theta1*d_theta5*cos(theta2)*cos(theta5)*sin(theta3))/4611686018427387904 + (5571380563941847*d_theta1*d_theta5*cos(theta3)*cos(theta5)*sin(theta2))/4611686018427387904 + (4653258611581729*d_theta1^2*cos(2*theta2)*sin(2*theta3)*sin(2*theta4)*cos(theta5))/36893488147419103232 + (4653258611581729*d_theta1^2*cos(2*theta3)*sin(2*theta2)*sin(2*theta4)*cos(theta5))/36893488147419103232 + (4653258611581729*d_theta1^2*cos(2*theta4)*sin(2*theta2)*sin(2*theta3)*cos(theta5))/36893488147419103232 + (1951319518623669*d_theta1*d_theta5*cos(theta2)*sin(theta3)*sin(theta4))/9223372036854775808 + (1951319518623669*d_theta1*d_theta5*cos(theta3)*sin(theta2)*sin(theta4))/9223372036854775808 + (1951319518623669*d_theta1*d_theta5*cos(theta4)*sin(theta2)*sin(theta3))/9223372036854775808 - (7988070105025833*d_theta1*d_theta5*cos(theta2)*sin(theta3)*sin(theta5))/2361183241434822606848 - (7988070105025833*d_theta1*d_theta5*cos(theta3)*sin(theta2)*sin(theta5))/2361183241434822606848 - (9004151162956663*d_theta1^2*cos(2*theta2)*sin(2*theta3)*sin(2*theta4)*sin(theta5))/18889465931478580854784 - (9004151162956663*d_theta1^2*cos(2*theta3)*sin(2*theta2)*sin(2*theta4)*sin(theta5))/18889465931478580854784 - (9004151162956663*d_theta1^2*cos(2*theta4)*sin(2*theta2)*sin(2*theta3)*sin(theta5))/18889465931478580854784 - (8313573984755043*d_theta1^2*cos(2*theta2)*cos(theta3)*cos(theta4)*cos(theta5))/18446744073709551616 + (5959870363491779*d_theta1^2*cos(2*theta2)*cos(theta3)*cos(theta4)*sin(theta5))/4722366482869645213696 + (3240011242931075*d_theta1*d_theta5*cos(2*theta5)*cos(theta2)*sin(theta3)*sin(theta4))/18446744073709551616 + (3240011242931075*d_theta1*d_theta5*cos(2*theta5)*cos(theta3)*sin(theta2)*sin(theta4))/18446744073709551616 + (3240011242931075*d_theta1*d_theta5*cos(2*theta5)*cos(theta4)*sin(theta2)*sin(theta3))/18446744073709551616 - (2282168433090971*d_theta1*d_theta5*sin(2*theta5)*cos(theta2)*sin(theta3)*sin(theta4))/9444732965739290427392 - (2282168433090971*d_theta1*d_theta5*sin(2*theta5)*cos(theta3)*sin(theta2)*sin(theta4))/9444732965739290427392 - (2282168433090971*d_theta1*d_theta5*sin(2*theta5)*cos(theta4)*sin(theta2)*sin(theta3))/9444732965739290427392 + (4653258611581729*d_theta1*d_theta5*cos(theta2)*cos(theta3)*cos(theta5)*sin(theta4))/18446744073709551616 + (4653258611581729*d_theta1*d_theta5*cos(theta2)*cos(theta4)*cos(theta5)*sin(theta3))/18446744073709551616 + (4653258611581729*d_theta1*d_theta5*cos(theta3)*cos(theta4)*cos(theta5)*sin(theta2))/18446744073709551616 - (9004151162956663*d_theta1*d_theta5*cos(theta2)*cos(theta3)*sin(theta4)*sin(theta5))/9444732965739290427392 - (9004151162956663*d_theta1*d_theta5*cos(theta2)*cos(theta4)*sin(theta3)*sin(theta5))/9444732965739290427392 - (9004151162956663*d_theta1*d_theta5*cos(theta3)*cos(theta4)*sin(theta2)*sin(theta5))/9444732965739290427392 - (4653258611581729*d_theta1*d_theta5*cos(theta5)*sin(theta2)*sin(theta3)*sin(theta4))/18446744073709551616 + (9004151162956663*d_theta1*d_theta5*sin(theta2)*sin(theta3)*sin(theta4)*sin(theta5))/9444732965739290427392 - (3240011242931075*d_theta1*d_theta5*cos(2*theta5)*cos(theta2)*cos(theta3)*cos(theta4))/18446744073709551616 + (2282168433090971*d_theta1*d_theta5*sin(2*theta5)*cos(theta2)*cos(theta3)*cos(theta4))/9444732965739290427392;
   (7220698343344529*d_theta1^2*sin(theta4))/4611686018427387904 - (d_theta1^2*sin(theta5))/5708990770823839524233143877797980545530986496 + (7220698343344529*d_theta2^2*sin(theta4))/2305843009213693952 + (7220698343344529*d_theta3^2*sin(theta4))/2305843009213693952 - (9004151162956663*d_theta5^2*sin(theta5))/18889465931478580854784 + (2787593*d_theta1^2*cos(2*theta4))/5575186299632655785383929568162090376495104 - (12544169*d_theta1^2*sin(2*theta4))/22300745198530623141535718272648361505980416 - (d_theta1^2*cos(theta5))/11150372599265311570767859136324180752990208 + (4653258611581729*d_theta5^2*cos(theta5))/36893488147419103232 + (7220698343344529*d_theta2*d_theta3*sin(theta4))/1152921504606846976 - (13937967*d_theta1^2*cos(2*theta2)*sin(theta4))/5575186299632655785383929568162090376495104 - (13937965*d_theta1^2*sin(2*theta2)*cos(theta4))/5575186299632655785383929568162090376495104 - (13937967*d_theta1^2*cos(2*theta3)*sin(theta4))/5575186299632655785383929568162090376495104 - (13937965*d_theta1^2*sin(2*theta3)*cos(theta4))/5575186299632655785383929568162090376495104 - (2854495*d_theta1^2*cos(2*theta4)*sin(theta5))/5708990770823839524233143877797980545530986496 - (2282168433090971*d_theta2*d_theta5*cos(2*theta5))/9444732965739290427392 - (2282168433090971*d_theta3*d_theta5*cos(2*theta5))/9444732965739290427392 - (2282168433090971*d_theta4*d_theta5*cos(2*theta5))/9444732965739290427392 - (3240011242931075*d_theta2*d_theta5*sin(2*theta5))/18446744073709551616 - (3240011242931075*d_theta3*d_theta5*sin(2*theta5))/18446744073709551616 - (3240011242931075*d_theta4*d_theta5*sin(2*theta5))/18446744073709551616 - (d_theta1^2*cos(2*theta4)*cos(2*theta5))/91343852333181432387730302044767688728495783936 - (11150375*d_theta1^2*cos(2*theta2)*sin(2*theta4))/178405961588244985132285746181186892047843328 + (89202975*d_theta1^2*cos(2*theta4)*sin(2*theta2))/178405961588244985132285746181186892047843328 - (11150375*d_theta1^2*cos(2*theta3)*sin(2*theta4))/178405961588244985132285746181186892047843328 + (89202975*d_theta1^2*cos(2*theta4)*sin(2*theta3))/178405961588244985132285746181186892047843328 - (1393797*d_theta1^2*cos(2*theta5)*sin(2*theta4))/22300745198530623141535718272648361505980416 - (17126969*d_theta1^2*sin(2*theta4)*sin(2*theta5))/91343852333181432387730302044767688728495783936 - (5571380563941847*d_theta1^2*cos(theta4)*cos(theta5))/18446744073709551616 - (5571380563941847*d_theta2^2*cos(theta4)*cos(theta5))/9223372036854775808 - (5571380563941847*d_theta3^2*cos(theta4)*cos(theta5))/9223372036854775808 + (5387337053181017*d_theta1^2*cos(theta3)*sin(theta4))/2305843009213693952 + (5387337053181017*d_theta1^2*cos(theta4)*sin(theta3))/2305843009213693952 + (5387337053181017*d_theta2^2*cos(theta3)*sin(theta4))/1152921504606846976 + (5387337053181017*d_theta2^2*cos(theta4)*sin(theta3))/1152921504606846976 + (7988070105025833*d_theta1^2*cos(theta4)*sin(theta5))/9444732965739290427392 + (7988070105025833*d_theta2^2*cos(theta4)*sin(theta5))/4722366482869645213696 + (7988070105025833*d_theta3^2*cos(theta4)*sin(theta5))/4722366482869645213696 + (5387337053181017*d_theta1^2*cos(2*theta2)*cos(theta3)*sin(theta4))/2305843009213693952 + (5387337053181017*d_theta1^2*cos(2*theta2)*cos(theta4)*sin(theta3))/2305843009213693952 + (5387337053181017*d_theta1^2*sin(2*theta2)*cos(theta3)*cos(theta4))/2305843009213693952 - (5387337053181017*d_theta1^2*sin(2*theta2)*sin(theta3)*sin(theta4))/2305843009213693952 + (7220698343344529*d_theta1^2*cos(2*theta2)*cos(2*theta3)*sin(theta4))/4611686018427387904 + (7220698343344529*d_theta1^2*cos(2*theta2)*sin(2*theta3)*cos(theta4))/4611686018427387904 + (7220698343344529*d_theta1^2*cos(2*theta3)*sin(2*theta2)*cos(theta4))/4611686018427387904 - (2854495*d_theta1^2*cos(2*theta2)*cos(2*theta4)*sin(theta5))/5708990770823839524233143877797980545530986496 - (2854495*d_theta1^2*cos(2*theta3)*cos(2*theta4)*sin(theta5))/5708990770823839524233143877797980545530986496 + (2787593*d_theta1^2*sin(2*theta2)*sin(2*theta4)*cos(theta5))/5575186299632655785383929568162090376495104 + (2787593*d_theta1^2*sin(2*theta3)*sin(2*theta4)*cos(theta5))/5575186299632655785383929568162090376495104 - (7220698343344529*d_theta1^2*sin(2*theta2)*sin(2*theta3)*sin(theta4))/4611686018427387904 - (8313573984755043*d_theta1^2*cos(theta3)*cos(theta4)*cos(theta5))/18446744073709551616 - (8313573984755043*d_theta2^2*cos(theta3)*cos(theta4)*cos(theta5))/9223372036854775808 + (5959870363491779*d_theta1^2*cos(theta3)*cos(theta4)*sin(theta5))/4722366482869645213696 + (5959870363491779*d_theta2^2*cos(theta3)*cos(theta4)*sin(theta5))/2361183241434822606848 + (2695991646372651*d_theta1^2*cos(2*theta2)*cos(2*theta3)*cos(2*theta4))/9223372036854775808 + (8313573984755043*d_theta1^2*cos(theta5)*sin(theta3)*sin(theta4))/18446744073709551616 + (8313573984755043*d_theta2^2*cos(theta5)*sin(theta3)*sin(theta4))/9223372036854775808 - (5571380563941847*d_theta2*d_theta3*cos(theta4)*cos(theta5))/4611686018427387904 + (1160499590055099*d_theta1^2*cos(2*theta2)*cos(2*theta3)*sin(2*theta4))/4611686018427387904 + (1160499590055099*d_theta1^2*cos(2*theta2)*cos(2*theta4)*sin(2*theta3))/4611686018427387904 + (1160499590055099*d_theta1^2*cos(2*theta3)*cos(2*theta4)*sin(2*theta2))/4611686018427387904 - (d_theta1^2*cos(2*theta2)*cos(2*theta4)*sin(2*theta5))/356811923176489970264571492362373784095686656 - (22300751*d_theta1^2*cos(2*theta2)*cos(2*theta5)*sin(2*theta4))/356811923176489970264571492362373784095686656 - (d_theta1^2*cos(2*theta4)*cos(2*theta5)*sin(2*theta2))/356811923176489970264571492362373784095686656 - (d_theta1^2*cos(2*theta3)*cos(2*theta4)*sin(2*theta5))/356811923176489970264571492362373784095686656 - (22300751*d_theta1^2*cos(2*theta3)*cos(2*theta5)*sin(2*theta4))/356811923176489970264571492362373784095686656 - (d_theta1^2*cos(2*theta4)*cos(2*theta5)*sin(2*theta3))/356811923176489970264571492362373784095686656 - (5959870363491779*d_theta1^2*sin(theta3)*sin(theta4)*sin(theta5))/4722366482869645213696 - (5959870363491779*d_theta2^2*sin(theta3)*sin(theta4)*sin(theta5))/2361183241434822606848 + (7988070105025833*d_theta2*d_theta3*cos(theta4)*sin(theta5))/2361183241434822606848 - (2695991646372651*d_theta1^2*cos(2*theta2)*sin(2*theta3)*sin(2*theta4))/9223372036854775808 - (2695991646372651*d_theta1^2*cos(2*theta3)*sin(2*theta2)*sin(2*theta4))/9223372036854775808 - (2695991646372651*d_theta1^2*cos(2*theta4)*sin(2*theta2)*sin(2*theta3))/9223372036854775808 - (2854495*d_theta1^2*cos(2*theta2)*sin(2*theta4)*sin(2*theta5))/45671926166590716193865151022383844364247891968 + (11417979*d_theta1^2*cos(2*theta4)*sin(2*theta2)*sin(2*theta5))/91343852333181432387730302044767688728495783936 - (d_theta1^2*cos(2*theta5)*sin(2*theta2)*sin(2*theta4))/91343852333181432387730302044767688728495783936 - (2854495*d_theta1^2*cos(2*theta3)*sin(2*theta4)*sin(2*theta5))/45671926166590716193865151022383844364247891968 + (11417979*d_theta1^2*cos(2*theta4)*sin(2*theta3)*sin(2*theta5))/91343852333181432387730302044767688728495783936 - (d_theta1^2*cos(2*theta5)*sin(2*theta3)*sin(2*theta4))/91343852333181432387730302044767688728495783936 - (1160499590055099*d_theta1^2*sin(2*theta2)*sin(2*theta3)*sin(2*theta4))/4611686018427387904 - (d_theta1^2*sin(2*theta2)*sin(2*theta4)*sin(2*theta5))/356811923176489970264571492362373784095686656 - (d_theta1^2*sin(2*theta3)*sin(2*theta4)*sin(2*theta5))/356811923176489970264571492362373784095686656 + (8313573984755043*d_theta1^2*cos(2*theta2)*cos(theta5)*sin(theta3)*sin(theta4))/18446744073709551616 + (8313573984755043*d_theta1^2*sin(2*theta2)*cos(theta3)*cos(theta5)*sin(theta4))/18446744073709551616 + (8313573984755043*d_theta1^2*sin(2*theta2)*cos(theta4)*cos(theta5)*sin(theta3))/18446744073709551616 - (3240011242931075*d_theta1^2*cos(2*theta2)*cos(2*theta3)*cos(2*theta5)*sin(2*theta4))/73786976294838206464 - (3240011242931075*d_theta1^2*cos(2*theta2)*cos(2*theta4)*cos(2*theta5)*sin(2*theta3))/73786976294838206464 - (3240011242931075*d_theta1^2*cos(2*theta3)*cos(2*theta4)*cos(2*theta5)*sin(2*theta2))/73786976294838206464 - (5959870363491779*d_theta1^2*cos(2*theta2)*sin(theta3)*sin(theta4)*sin(theta5))/4722366482869645213696 - (5959870363491779*d_theta1^2*sin(2*theta2)*cos(theta3)*sin(theta4)*sin(theta5))/4722366482869645213696 - (5959870363491779*d_theta1^2*sin(2*theta2)*cos(theta4)*sin(theta3)*sin(theta5))/4722366482869645213696 + (2282168433090971*d_theta1^2*cos(2*theta2)*cos(2*theta3)*sin(2*theta4)*sin(2*theta5))/37778931862957161709568 + (2282168433090971*d_theta1^2*cos(2*theta2)*cos(2*theta4)*sin(2*theta3)*sin(2*theta5))/37778931862957161709568 + (2282168433090971*d_theta1^2*cos(2*theta3)*cos(2*theta4)*sin(2*theta2)*sin(2*theta5))/37778931862957161709568 + (3240011242931075*d_theta1^2*cos(2*theta5)*sin(2*theta2)*sin(2*theta3)*sin(2*theta4))/73786976294838206464 - (2282168433090971*d_theta1^2*sin(2*theta2)*sin(2*theta3)*sin(2*theta4)*sin(2*theta5))/37778931862957161709568 - (5571380563941847*d_theta1^2*cos(2*theta2)*cos(2*theta3)*cos(theta4)*cos(theta5))/18446744073709551616 + (7988070105025833*d_theta1^2*cos(2*theta2)*cos(2*theta3)*cos(theta4)*sin(theta5))/9444732965739290427392 + (5571380563941847*d_theta1^2*cos(2*theta2)*sin(2*theta3)*cos(theta5)*sin(theta4))/18446744073709551616 + (5571380563941847*d_theta1^2*cos(2*theta3)*sin(2*theta2)*cos(theta5)*sin(theta4))/18446744073709551616 + (5571380563941847*d_theta1^2*sin(2*theta2)*sin(2*theta3)*cos(theta4)*cos(theta5))/18446744073709551616 - (7988070105025833*d_theta1^2*cos(2*theta2)*sin(2*theta3)*sin(theta4)*sin(theta5))/9444732965739290427392 - (7988070105025833*d_theta1^2*cos(2*theta3)*sin(2*theta2)*sin(theta4)*sin(theta5))/9444732965739290427392 - (7988070105025833*d_theta1^2*sin(2*theta2)*sin(2*theta3)*cos(theta4)*sin(theta5))/9444732965739290427392 - (4653258611581729*d_theta1^2*cos(2*theta2)*cos(2*theta3)*cos(2*theta4)*cos(theta5))/36893488147419103232 - (1951319518623669*d_theta1*d_theta5*cos(theta2)*cos(theta3)*cos(theta4))/9223372036854775808 + (9004151162956663*d_theta1^2*cos(2*theta2)*cos(2*theta3)*cos(2*theta4)*sin(theta5))/18889465931478580854784 + (4653258611581729*d_theta1^2*cos(2*theta2)*sin(2*theta3)*sin(2*theta4)*cos(theta5))/36893488147419103232 + (4653258611581729*d_theta1^2*cos(2*theta3)*sin(2*theta2)*sin(2*theta4)*cos(theta5))/36893488147419103232 + (4653258611581729*d_theta1^2*cos(2*theta4)*sin(2*theta2)*sin(2*theta3)*cos(theta5))/36893488147419103232 + (1951319518623669*d_theta1*d_theta5*cos(theta2)*sin(theta3)*sin(theta4))/9223372036854775808 + (1951319518623669*d_theta1*d_theta5*cos(theta3)*sin(theta2)*sin(theta4))/9223372036854775808 + (1951319518623669*d_theta1*d_theta5*cos(theta4)*sin(theta2)*sin(theta3))/9223372036854775808 - (9004151162956663*d_theta1^2*cos(2*theta2)*sin(2*theta3)*sin(2*theta4)*sin(theta5))/18889465931478580854784 - (9004151162956663*d_theta1^2*cos(2*theta3)*sin(2*theta2)*sin(2*theta4)*sin(theta5))/18889465931478580854784 - (9004151162956663*d_theta1^2*cos(2*theta4)*sin(2*theta2)*sin(2*theta3)*sin(theta5))/18889465931478580854784 - (8313573984755043*d_theta1^2*cos(2*theta2)*cos(theta3)*cos(theta4)*cos(theta5))/18446744073709551616 + (5959870363491779*d_theta1^2*cos(2*theta2)*cos(theta3)*cos(theta4)*sin(theta5))/4722366482869645213696 + (3240011242931075*d_theta1*d_theta5*cos(2*theta5)*cos(theta2)*sin(theta3)*sin(theta4))/18446744073709551616 + (3240011242931075*d_theta1*d_theta5*cos(2*theta5)*cos(theta3)*sin(theta2)*sin(theta4))/18446744073709551616 + (3240011242931075*d_theta1*d_theta5*cos(2*theta5)*cos(theta4)*sin(theta2)*sin(theta3))/18446744073709551616 - (2282168433090971*d_theta1*d_theta5*sin(2*theta5)*cos(theta2)*sin(theta3)*sin(theta4))/9444732965739290427392 - (2282168433090971*d_theta1*d_theta5*sin(2*theta5)*cos(theta3)*sin(theta2)*sin(theta4))/9444732965739290427392 - (2282168433090971*d_theta1*d_theta5*sin(2*theta5)*cos(theta4)*sin(theta2)*sin(theta3))/9444732965739290427392 + (4653258611581729*d_theta1*d_theta5*cos(theta2)*cos(theta3)*cos(theta5)*sin(theta4))/18446744073709551616 + (4653258611581729*d_theta1*d_theta5*cos(theta2)*cos(theta4)*cos(theta5)*sin(theta3))/18446744073709551616 + (4653258611581729*d_theta1*d_theta5*cos(theta3)*cos(theta4)*cos(theta5)*sin(theta2))/18446744073709551616 - (9004151162956663*d_theta1*d_theta5*cos(theta2)*cos(theta3)*sin(theta4)*sin(theta5))/9444732965739290427392 - (9004151162956663*d_theta1*d_theta5*cos(theta2)*cos(theta4)*sin(theta3)*sin(theta5))/9444732965739290427392 - (9004151162956663*d_theta1*d_theta5*cos(theta3)*cos(theta4)*sin(theta2)*sin(theta5))/9444732965739290427392 - (4653258611581729*d_theta1*d_theta5*cos(theta5)*sin(theta2)*sin(theta3)*sin(theta4))/18446744073709551616 + (9004151162956663*d_theta1*d_theta5*sin(theta2)*sin(theta3)*sin(theta4)*sin(theta5))/9444732965739290427392 - (3240011242931075*d_theta1*d_theta5*cos(2*theta5)*cos(theta2)*cos(theta3)*cos(theta4))/18446744073709551616 + (2282168433090971*d_theta1*d_theta5*sin(2*theta5)*cos(theta2)*cos(theta3)*cos(theta4))/9444732965739290427392;
   (5959870363491779*d_theta1^2*sin(2*theta2 + theta3 + theta4 + theta5))/9444732965739290427392 - (2854495*d_theta1^2*sin(2*theta2 + 2*theta4 + theta5))/22835963083295358096932575511191922182123945984 - (2854495*d_theta1^2*sin(2*theta3 + 2*theta4 + theta5))/22835963083295358096932575511191922182123945984 - (8313573984755043*d_theta1^2*cos(2*theta2 + theta3 + theta4 + theta5))/36893488147419103232 - (2854495*d_theta1^2*sin(2*theta2 + 2*theta3 + theta5))/22835963083295358096932575511191922182123945984 + (5571380563941847*d_theta1^2*cos(theta4 - theta5))/36893488147419103232 + (5571380563941847*d_theta2^2*cos(theta4 - theta5))/18446744073709551616 + (5571380563941847*d_theta3^2*cos(theta4 - theta5))/18446744073709551616 + (4653258611581729*d_theta1^2*cos(2*theta2 + 2*theta3 + 2*theta4 - theta5))/147573952589676412928 - (2282168433090971*d_theta1^2*cos(2*theta2 + 2*theta3 + 2*theta4 - 2*theta5))/75557863725914323419136 - (2282168433090971*d_theta1^2*cos(2*theta2 + 2*theta3 + 2*theta4 + 2*theta5))/75557863725914323419136 - (2854495*d_theta1^2*sin(2*theta2 + theta5))/22835963083295358096932575511191922182123945984 + (7988070105025833*d_theta1^2*sin(theta4 - theta5))/18889465931478580854784 - (2854495*d_theta1^2*sin(2*theta3 + theta5))/22835963083295358096932575511191922182123945984 - (2854495*d_theta1^2*sin(2*theta4 + theta5))/22835963083295358096932575511191922182123945984 + (7988070105025833*d_theta2^2*sin(theta4 - theta5))/9444732965739290427392 + (7988070105025833*d_theta3^2*sin(theta4 - theta5))/9444732965739290427392 - (8313573984755043*d_theta1^2*cos(theta3 + theta4 + theta5))/36893488147419103232 - (8313573984755043*d_theta2^2*cos(theta3 + theta4 + theta5))/18446744073709551616 + (9004151162956663*d_theta1^2*sin(2*theta2 + 2*theta3 + 2*theta4 - theta5))/75557863725914323419136 + (3240011242931075*d_theta1^2*sin(2*theta2 + 2*theta3 + 2*theta4 - 2*theta5))/147573952589676412928 - (3240011242931075*d_theta1^2*sin(2*theta2 + 2*theta3 + 2*theta4 + 2*theta5))/147573952589676412928 + (5959870363491779*d_theta1^2*sin(theta3 + theta4 + theta5))/9444732965739290427392 + (5959870363491779*d_theta2^2*sin(theta3 + theta4 + theta5))/4722366482869645213696 - (d_theta1^2*cos(2*theta2))/22835963083295358096932575511191922182123945984 - (d_theta1^2*cos(2*theta3))/22835963083295358096932575511191922182123945984 - (d_theta1^2*cos(2*theta4))/22835963083295358096932575511191922182123945984 - (2282168433090971*d_theta1^2*cos(2*theta5))/37778931862957161709568 + (2282168433090971*d_theta2^2*cos(2*theta5))/18889465931478580854784 + (2282168433090971*d_theta3^2*cos(2*theta5))/18889465931478580854784 + (2282168433090971*d_theta4^2*cos(2*theta5))/18889465931478580854784 - (2854495*d_theta1^2*cos(2*theta2 + 2*theta3 - 2*theta5))/45671926166590716193865151022383844364247891968 - (2854495*d_theta1^2*cos(2*theta2 + 2*theta3 + 2*theta5))/45671926166590716193865151022383844364247891968 - (2854495*d_theta1^2*cos(2*theta2 + 2*theta4 - 2*theta5))/45671926166590716193865151022383844364247891968 - (2854495*d_theta1^2*cos(2*theta2 + 2*theta4 + 2*theta5))/45671926166590716193865151022383844364247891968 - (2854495*d_theta1^2*cos(2*theta3 + 2*theta4 - 2*theta5))/45671926166590716193865151022383844364247891968 - (2854495*d_theta1^2*cos(2*theta3 + 2*theta4 + 2*theta5))/45671926166590716193865151022383844364247891968 - (3240011242931075*d_theta1^2*sin(2*theta5))/73786976294838206464 + (3240011242931075*d_theta2^2*sin(2*theta5))/36893488147419103232 + (3240011242931075*d_theta3^2*sin(2*theta5))/36893488147419103232 + (3240011242931075*d_theta4^2*sin(2*theta5))/36893488147419103232 - (2854495*d_theta1^2*sin(2*theta2 + 2*theta3 - theta5))/22835963083295358096932575511191922182123945984 - (d_theta1^2*sin(2*theta3 - 2*theta2 + 2*theta5))/356811923176489970264571492362373784095686656 - (d_theta1^2*sin(2*theta2 - 2*theta3 + 2*theta5))/356811923176489970264571492362373784095686656 + (5575187*d_theta1^2*sin(2*theta2 + 2*theta3 - 2*theta5))/178405961588244985132285746181186892047843328 - (5575187*d_theta1^2*sin(2*theta2 + 2*theta3 + 2*theta5))/178405961588244985132285746181186892047843328 - (2854495*d_theta1^2*sin(2*theta2 + 2*theta4 - theta5))/22835963083295358096932575511191922182123945984 - (d_theta1^2*sin(2*theta4 - 2*theta2 + 2*theta5))/356811923176489970264571492362373784095686656 - (d_theta1^2*sin(2*theta2 - 2*theta4 + 2*theta5))/356811923176489970264571492362373784095686656 + (5575187*d_theta1^2*sin(2*theta2 + 2*theta4 - 2*theta5))/178405961588244985132285746181186892047843328 - (5575187*d_theta1^2*sin(2*theta2 + 2*theta4 + 2*theta5))/178405961588244985132285746181186892047843328 - (2854495*d_theta1^2*sin(2*theta3 + 2*theta4 - theta5))/22835963083295358096932575511191922182123945984 - (d_theta1^2*sin(2*theta4 - 2*theta3 + 2*theta5))/356811923176489970264571492362373784095686656 - (d_theta1^2*sin(2*theta3 - 2*theta4 + 2*theta5))/356811923176489970264571492362373784095686656 + (5575187*d_theta1^2*sin(2*theta3 + 2*theta4 - 2*theta5))/178405961588244985132285746181186892047843328 - (5575187*d_theta1^2*sin(2*theta3 + 2*theta4 + 2*theta5))/178405961588244985132285746181186892047843328 + (8313573984755043*d_theta1^2*cos(2*theta2 + theta3 + theta4 - theta5))/36893488147419103232 - (5571380563941847*d_theta1^2*cos(2*theta2 + 2*theta3 + theta4 + theta5))/36893488147419103232 + (5959870363491779*d_theta1^2*sin(2*theta2 + theta3 + theta4 - theta5))/9444732965739290427392 + (7988070105025833*d_theta1^2*sin(2*theta2 + 2*theta3 + theta4 + theta5))/18889465931478580854784 - (2854495*d_theta1^2*cos(2*theta2 - 2*theta5))/45671926166590716193865151022383844364247891968 - (2854495*d_theta1^2*cos(2*theta2 + 2*theta5))/45671926166590716193865151022383844364247891968 - (2854495*d_theta1^2*cos(2*theta3 - 2*theta5))/45671926166590716193865151022383844364247891968 - (2854495*d_theta1^2*cos(2*theta3 + 2*theta5))/45671926166590716193865151022383844364247891968 - (2854495*d_theta1^2*cos(2*theta4 - 2*theta5))/45671926166590716193865151022383844364247891968 - (2854495*d_theta1^2*cos(2*theta4 + 2*theta5))/45671926166590716193865151022383844364247891968 - (2854495*d_theta1^2*sin(2*theta2 - theta5))/22835963083295358096932575511191922182123945984 + (5575187*d_theta1^2*sin(2*theta2 - 2*theta5))/178405961588244985132285746181186892047843328 - (1393797*d_theta1^2*sin(2*theta2 + 2*theta5))/44601490397061246283071436545296723011960832 - (2854495*d_theta1^2*sin(2*theta3 - theta5))/22835963083295358096932575511191922182123945984 + (5575187*d_theta1^2*sin(2*theta3 - 2*theta5))/178405961588244985132285746181186892047843328 - (1393797*d_theta1^2*sin(2*theta3 + 2*theta5))/44601490397061246283071436545296723011960832 - (2854495*d_theta1^2*sin(2*theta4 - theta5))/22835963083295358096932575511191922182123945984 + (5575187*d_theta1^2*sin(2*theta4 - 2*theta5))/178405961588244985132285746181186892047843328 - (1393797*d_theta1^2*sin(2*theta4 + 2*theta5))/44601490397061246283071436545296723011960832 + (8313573984755043*d_theta1^2*cos(theta3 + theta4 - theta5))/36893488147419103232 + (8313573984755043*d_theta2^2*cos(theta3 + theta4 - theta5))/18446744073709551616 + (5959870363491779*d_theta1^2*sin(theta3 + theta4 - theta5))/9444732965739290427392 + (5959870363491779*d_theta2^2*sin(theta3 + theta4 - theta5))/4722366482869645213696 - d_theta1^2/22835963083295358096932575511191922182123945984 - (5571380563941847*d_theta1^2*cos(theta4 + theta5))/36893488147419103232 - (5571380563941847*d_theta2^2*cos(theta4 + theta5))/18446744073709551616 - (5571380563941847*d_theta3^2*cos(theta4 + theta5))/18446744073709551616 + (5571380563941847*d_theta1^2*cos(2*theta2 + 2*theta3 + theta4 - theta5))/36893488147419103232 - (4653258611581729*d_theta1^2*cos(2*theta2 + 2*theta3 + 2*theta4 + theta5))/147573952589676412928 + (7988070105025833*d_theta1^2*sin(theta4 + theta5))/18889465931478580854784 + (7988070105025833*d_theta2^2*sin(theta4 + theta5))/9444732965739290427392 + (7988070105025833*d_theta3^2*sin(theta4 + theta5))/9444732965739290427392 + (7988070105025833*d_theta1^2*sin(2*theta2 + 2*theta3 + theta4 - theta5))/18889465931478580854784 + (9004151162956663*d_theta1^2*sin(2*theta2 + 2*theta3 + 2*theta4 + theta5))/75557863725914323419136 + (9004151162956663*d_theta1*d_theta2*cos(theta2 + theta3 + theta4 - theta5))/18889465931478580854784 + (3240011242931075*d_theta1*d_theta2*cos(theta2 + theta3 + theta4 - 2*theta5))/36893488147419103232 + (3240011242931075*d_theta1*d_theta2*cos(theta2 + theta3 + theta4 + 2*theta5))/36893488147419103232 + (9004151162956663*d_theta1*d_theta3*cos(theta2 + theta3 + theta4 - theta5))/18889465931478580854784 + (3240011242931075*d_theta1*d_theta3*cos(theta2 + theta3 + theta4 - 2*theta5))/36893488147419103232 + (3240011242931075*d_theta1*d_theta3*cos(theta2 + theta3 + theta4 + 2*theta5))/36893488147419103232 + (9004151162956663*d_theta1*d_theta4*cos(theta2 + theta3 + theta4 - theta5))/18889465931478580854784 + (3240011242931075*d_theta1*d_theta4*cos(theta2 + theta3 + theta4 - 2*theta5))/36893488147419103232 + (3240011242931075*d_theta1*d_theta4*cos(theta2 + theta3 + theta4 + 2*theta5))/36893488147419103232 - (4653258611581729*d_theta1*d_theta2*sin(theta2 + theta3 + theta4 - theta5))/36893488147419103232 + (2282168433090971*d_theta1*d_theta2*sin(theta2 + theta3 + theta4 - 2*theta5))/18889465931478580854784 - (2282168433090971*d_theta1*d_theta2*sin(theta2 + theta3 + theta4 + 2*theta5))/18889465931478580854784 - (4653258611581729*d_theta1*d_theta3*sin(theta2 + theta3 + theta4 - theta5))/36893488147419103232 + (2282168433090971*d_theta1*d_theta3*sin(theta2 + theta3 + theta4 - 2*theta5))/18889465931478580854784 - (2282168433090971*d_theta1*d_theta3*sin(theta2 + theta3 + theta4 + 2*theta5))/18889465931478580854784 - (4653258611581729*d_theta1*d_theta4*sin(theta2 + theta3 + theta4 - theta5))/36893488147419103232 + (2282168433090971*d_theta1*d_theta4*sin(theta2 + theta3 + theta4 - 2*theta5))/18889465931478580854784 - (2282168433090971*d_theta1*d_theta4*sin(theta2 + theta3 + theta4 + 2*theta5))/18889465931478580854784 + (5959870363491779*d_theta1*d_theta2*cos(theta2 - theta5))/2361183241434822606848 + (5571380563941847*d_theta2*d_theta3*cos(theta4 - theta5))/9223372036854775808 - (8313573984755043*d_theta1*d_theta2*sin(theta2 - theta5))/9223372036854775808 + (7988070105025833*d_theta2*d_theta3*sin(theta4 - theta5))/4722366482869645213696 + (1951319518623669*d_theta1*d_theta2*cos(theta2 + theta3 + theta4))/9223372036854775808 - (7988070105025833*d_theta1*d_theta2*cos(theta2 + theta3 + theta5))/4722366482869645213696 + (1951319518623669*d_theta1*d_theta3*cos(theta2 + theta3 + theta4))/9223372036854775808 - (7988070105025833*d_theta1*d_theta3*cos(theta2 + theta3 + theta5))/4722366482869645213696 + (1951319518623669*d_theta1*d_theta4*cos(theta2 + theta3 + theta4))/9223372036854775808 - (5571380563941847*d_theta1*d_theta2*sin(theta2 + theta3 + theta5))/9223372036854775808 - (5571380563941847*d_theta1*d_theta3*sin(theta2 + theta3 + theta5))/9223372036854775808 + (2282168433090971*d_theta2*d_theta3*cos(2*theta5))/9444732965739290427392 + (2282168433090971*d_theta2*d_theta4*cos(2*theta5))/9444732965739290427392 + (2282168433090971*d_theta3*d_theta4*cos(2*theta5))/9444732965739290427392 + (3240011242931075*d_theta2*d_theta3*sin(2*theta5))/18446744073709551616 + (3240011242931075*d_theta2*d_theta4*sin(2*theta5))/18446744073709551616 + (3240011242931075*d_theta3*d_theta4*sin(2*theta5))/18446744073709551616 + (7988070105025833*d_theta1*d_theta2*cos(theta2 + theta3 - theta5))/4722366482869645213696 + (7988070105025833*d_theta1*d_theta3*cos(theta2 + theta3 - theta5))/4722366482869645213696 - (5571380563941847*d_theta1*d_theta2*sin(theta2 + theta3 - theta5))/9223372036854775808 - (5571380563941847*d_theta1*d_theta3*sin(theta2 + theta3 - theta5))/9223372036854775808 - (9004151162956663*d_theta1*d_theta2*cos(theta2 + theta3 + theta4 + theta5))/18889465931478580854784 - (9004151162956663*d_theta1*d_theta3*cos(theta2 + theta3 + theta4 + theta5))/18889465931478580854784 - (9004151162956663*d_theta1*d_theta4*cos(theta2 + theta3 + theta4 + theta5))/18889465931478580854784 - (4653258611581729*d_theta1*d_theta2*sin(theta2 + theta3 + theta4 + theta5))/36893488147419103232 - (4653258611581729*d_theta1*d_theta3*sin(theta2 + theta3 + theta4 + theta5))/36893488147419103232 - (4653258611581729*d_theta1*d_theta4*sin(theta2 + theta3 + theta4 + theta5))/36893488147419103232 - (5959870363491779*d_theta1*d_theta2*cos(theta2 + theta5))/2361183241434822606848 - (5571380563941847*d_theta2*d_theta3*cos(theta4 + theta5))/9223372036854775808 - (8313573984755043*d_theta1*d_theta2*sin(theta2 + theta5))/9223372036854775808 + (7988070105025833*d_theta2*d_theta3*sin(theta4 + theta5))/4722366482869645213696];
y = Z;
